simulink model "Model"  (R2016a)
settings: Solver=VariableStepAuto  StartTime=0.0  StopTime=0  RelTol=1e-3
values from neighbouring files (symbols this model uses):
  disdef = variable(a, 7)    [CollectionAG806_808.m]
  Dpha = 0    [CollectionAG806_808.m]    (also in CourantCCabc.m)
  Dphb = -120    [CollectionAG806_808.m]    (also in CourantCCabc.m)
  Dphc = +120    (= 120)    [CollectionAG806_808.m]    (also in CourantCCabc.m)
  frequence = 60    [CollectionAG806_808.m]    (also in CourantCCabc.m)
  Qc844 = [100e3 100e3 100e3]    [CollectionAG806_808.m]    (also in CourantCCabc.m)
  Qc848 = [150e3 150e3 150e3]    [CollectionAG806_808.m]    (also in CourantCCabc.m)
  RF1 = variable(a, 6)    [CollectionAG806_808.m]
  Ustation = variable(a, 2)    [CollectionAG806_808.m]
  Vstation = variable(a, 1)    [CollectionAG806_808.m]
undefined symbols (not defined in the file or in its folder): activeA, activeB, activeC, C_300, C_301, C_302, C_303, C_304, L_300, L_301, L_302, L_303, L_304, Ltot_806_808, R_300, R_301, R_302, R_303, R_304, reactiveA, reactiveB, reactiveC
libraries: powerlib x311
(part 1 of 2)
settings Model: Creator=HP  LastModifiedBy=HP

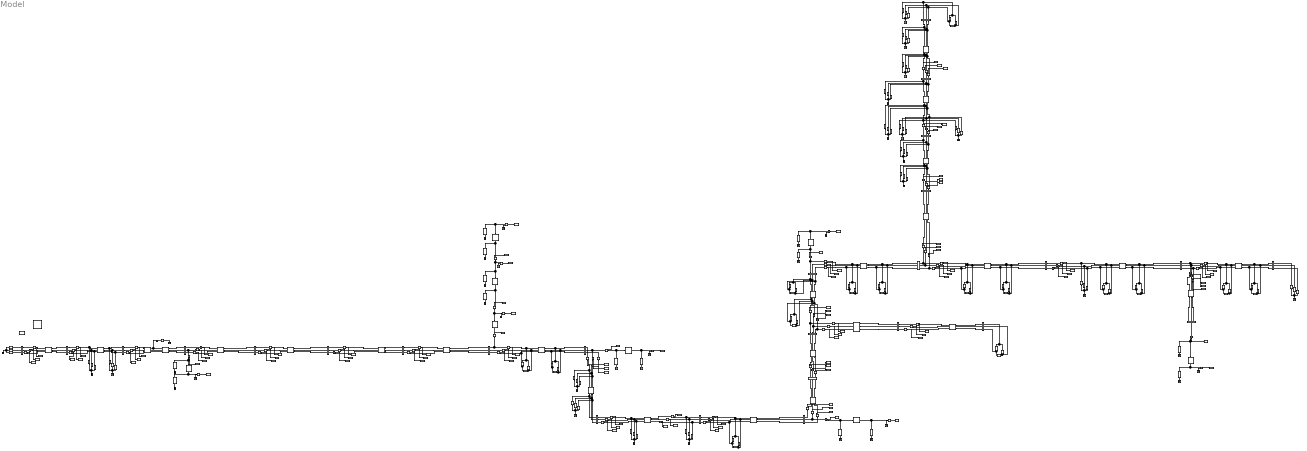
== system Model ==
  "800 " : powerlib/Measurements/Three-Phase V-I Measurement  VoltageMeasurement=phase-to-ground  SetLabelV=on  LabelV=V800  Vpu=off  VpuLL=off  CurrentMeasurement=no  SetLabelI=on  LabelI=I800_802  Ipu=off  Pbase=100e6  Vbase=500e3  OutputType=Complex  PhasorSimulation=on  PSBequivalent=0
  "802 " : powerlib/Measurements/Three-Phase V-I Measurement  VoltageMeasurement=phase-to-ground  SetLabelV=on  LabelV=V802  Vpu=off  VpuLL=off  CurrentMeasurement=no  SetLabelI=on  LabelI=I802_806  Ipu=off  Pbase=100e6  Vbase=500e3  OutputType=Complex  PhasorSimulation=on  PSBequivalent=0
  806 : powerlib/Measurements/Three-Phase V-I Measurement  VoltageMeasurement=phase-to-ground  SetLabelV=on  LabelV=V806  Vpu=off  VpuLL=off  CurrentMeasurement=no  SetLabelI=on  LabelI=I806_808  Ipu=off  Pbase=100e6  Vbase=500e3  OutputType=Complex  PhasorSimulation=on  PSBequivalent=0
  808 : powerlib/Measurements/Three-Phase V-I Measurement  VoltageMeasurement=phase-to-ground  SetLabelV=on  LabelV=V808  Vpu=off  VpuLL=off  CurrentMeasurement=no  SetLabelI=on  LabelI=I808_810_812  Ipu=off  Pbase=100e6  Vbase=500e3  OutputType=Complex  PhasorSimulation=on  PSBequivalent=0
  812 : powerlib/Measurements/Three-Phase V-I Measurement  VoltageMeasurement=phase-to-ground  SetLabelV=on  LabelV=V812  Vpu=off  VpuLL=off  CurrentMeasurement=no  SetLabelI=on  LabelI=I812_814  Ipu=off  Pbase=100e6  Vbase=500e3  OutputType=Complex  PhasorSimulation=on  PSBequivalent=0
  814 : powerlib/Measurements/Three-Phase V-I Measurement  VoltageMeasurement=phase-to-ground  SetLabelV=on  LabelV=V814  Vpu=off  VpuLL=off  CurrentMeasurement=no  SetLabelI=on  LabelI=I814_850  Ipu=off  Pbase=100e6  Vbase=500e3  OutputType=Complex  PhasorSimulation=on  PSBequivalent=0
  816 : powerlib/Measurements/Three-Phase V-I Measurement  VoltageMeasurement=phase-to-ground  SetLabelV=on  LabelV=V816  Vpu=off  VpuLL=off  CurrentMeasurement=no  SetLabelI=on  LabelI=I816_818_824  Ipu=off  Pbase=100e6  Vbase=500e3  OutputType=Complex  PhasorSimulation=on  PSBequivalent=0
  824 : powerlib/Measurements/Three-Phase V-I Measurement  VoltageMeasurement=phase-to-ground  SetLabelV=on  LabelV=V824  Vpu=off  VpuLL=off  CurrentMeasurement=no  SetLabelI=on  LabelI=I824_826_828  Ipu=off  Pbase=100e6  Vbase=500e3  OutputType=Complex  PhasorSimulation=on  PSBequivalent=0
  828 : powerlib/Measurements/Three-Phase V-I Measurement  VoltageMeasurement=phase-to-ground  SetLabelV=on  LabelV=V828  Vpu=off  VpuLL=off  CurrentMeasurement=no  SetLabelI=on  LabelI=I828_830  Ipu=off  Pbase=100e6  Vbase=500e3  OutputType=Complex  PhasorSimulation=on  PSBequivalent=0
  830 : powerlib/Measurements/Three-Phase V-I Measurement  VoltageMeasurement=phase-to-ground  SetLabelV=on  LabelV=V830  Vpu=off  VpuLL=off  CurrentMeasurement=no  SetLabelI=on  LabelI=I830_854  Ipu=off  Pbase=100e6  Vbase=500e3  OutputType=Complex  PhasorSimulation=on  PSBequivalent=0
  832 : powerlib/Measurements/Three-Phase V-I Measurement  VoltageMeasurement=phase-to-ground  SetLabelV=on  LabelV=V832  Vpu=off  VpuLL=off  CurrentMeasurement=no  SetLabelI=on  LabelI=I832_858_888  Ipu=off  Pbase=100e6  Vbase=500e3  OutputType=Complex  PhasorSimulation=on  PSBequivalent=0
  834 : powerlib/Measurements/Three-Phase V-I Measurement  VoltageMeasurement=phase-to-ground  SetLabelV=on  LabelV=V834  Vpu=off  VpuLL=off  CurrentMeasurement=no  SetLabelI=off  LabelI=I834_842_860  Ipu=off  Pbase=100e6  Vbase=500e3  OutputType=Complex  PhasorSimulation=on  PSBequivalent=0
  836 : powerlib/Measurements/Three-Phase V-I Measurement  VoltageMeasurement=phase-to-ground  SetLabelV=on  LabelV=V836  Vpu=off  VpuLL=off  CurrentMeasurement=no  SetLabelI=off  LabelI=Iabc  Ipu=off  Pbase=100e6  Vbase=500e3  OutputType=Complex  PhasorSimulation=on  PSBequivalent=0
  840 : powerlib/Measurements/Three-Phase V-I Measurement  VoltageMeasurement=phase-to-ground  SetLabelV=on  LabelV=V840  Vpu=off  VpuLL=off  CurrentMeasurement=no  SetLabelI=on  LabelI=Iabc  Ipu=off  Pbase=100e6  Vbase=500e3  OutputType=Complex  PhasorSimulation=on  PSBequivalent=0
  842 : powerlib/Measurements/Three-Phase V-I Measurement  VoltageMeasurement=phase-to-ground  SetLabelV=on  LabelV=V842  Vpu=off  VpuLL=off  CurrentMeasurement=no  SetLabelI=on  LabelI=I842_844  Ipu=off  Pbase=100e6  Vbase=500e3  OutputType=Complex  PhasorSimulation=on  PSBequivalent=0
  844 : powerlib/Measurements/Three-Phase V-I Measurement  VoltageMeasurement=phase-to-ground  SetLabelV=on  LabelV=V844  Vpu=off  VpuLL=off  CurrentMeasurement=no  SetLabelI=on  LabelI=I844_846  Ipu=off  Pbase=100e6  Vbase=500e3  OutputType=Complex  PhasorSimulation=on  PSBequivalent=0
  846 : powerlib/Measurements/Three-Phase V-I Measurement  VoltageMeasurement=phase-to-ground  SetLabelV=on  LabelV=V846  Vpu=off  VpuLL=off  CurrentMeasurement=no  SetLabelI=on  LabelI=I846_848  Ipu=off  Pbase=100e6  Vbase=500e3  OutputType=Complex  PhasorSimulation=on  PSBequivalent=0
  848 : powerlib/Measurements/Three-Phase V-I Measurement  VoltageMeasurement=phase-to-ground  SetLabelV=on  LabelV=V848  Vpu=off  VpuLL=off  CurrentMeasurement=no  SetLabelI=on  LabelI=I846_848  Ipu=off  Pbase=100e6  Vbase=500e3  OutputType=Complex  PhasorSimulation=on  PSBequivalent=0
  850 : powerlib/Measurements/Three-Phase V-I Measurement  VoltageMeasurement=phase-to-ground  SetLabelV=on  LabelV=V850  Vpu=off  VpuLL=off  CurrentMeasurement=no  SetLabelI=on  LabelI=I850_816  Ipu=off  Pbase=100e6  Vbase=500e3  OutputType=Complex  PhasorSimulation=on  PSBequivalent=0
  852 : powerlib/Measurements/Three-Phase V-I Measurement  VoltageMeasurement=phase-to-ground  SetLabelV=on  LabelV=V852  Vpu=off  VpuLL=off  CurrentMeasurement=no  SetLabelI=on  LabelI=I852_832  Ipu=off  Pbase=100e6  Vbase=500e3  OutputType=Complex  PhasorSimulation=on  PSBequivalent=0
  854 : powerlib/Measurements/Three-Phase V-I Measurement  VoltageMeasurement=phase-to-ground  SetLabelV=on  LabelV=V854  Vpu=off  VpuLL=off  CurrentMeasurement=no  SetLabelI=on  LabelI=I854_852_856  Ipu=off  Pbase=100e6  Vbase=500e3  OutputType=Complex  PhasorSimulation=on  PSBequivalent=0
  858 : powerlib/Measurements/Three-Phase V-I Measurement  VoltageMeasurement=phase-to-ground  SetLabelV=on  LabelV=V858  Vpu=off  VpuLL=off  CurrentMeasurement=no  SetLabelI=on  LabelI=I858_834_864  Ipu=off  Pbase=100e6  Vbase=500e3  OutputType=Complex  PhasorSimulation=on  PSBequivalent=0
  860 : powerlib/Measurements/Three-Phase V-I Measurement  VoltageMeasurement=phase-to-ground  SetLabelV=on  LabelV=V860  Vpu=off  VpuLL=off  CurrentMeasurement=no  SetLabelI=on  LabelI=I860_836  Ipu=off  Pbase=100e6  Vbase=500e3  OutputType=Complex  PhasorSimulation=on  PSBequivalent=0
  862 : powerlib/Measurements/Three-Phase V-I Measurement  VoltageMeasurement=phase-to-ground  SetLabelV=on  LabelV=V862  Vpu=off  VpuLL=off  CurrentMeasurement=no  SetLabelI=on  LabelI=Iabc  Ipu=off  Pbase=100e6  Vbase=500e3  OutputType=Complex  PhasorSimulation=on  PSBequivalent=0
  888 : powerlib/Measurements/Three-Phase V-I Measurement  VoltageMeasurement=phase-to-ground  SetLabelV=on  LabelV=V888  Vpu=off  VpuLL=off  CurrentMeasurement=no  SetLabelI=on  LabelI=I888_890  Ipu=off  Pbase=100e6  Vbase=500e3  OutputType=Complex  PhasorSimulation=on  PSBequivalent=0
  890 : powerlib/Measurements/Three-Phase V-I Measurement  VoltageMeasurement=phase-to-ground  SetLabelV=on  LabelV=V890  Vpu=off  VpuLL=off  CurrentMeasurement=no  SetLabelI=on  LabelI=I888_890  Ipu=off  Pbase=100e6  Vbase=500e3  OutputType=Complex  PhasorSimulation=on  PSBequivalent=0
  Breaker : powerlib/Elements/Breaker  InitialState=0  SwitchingTimes=0  External=off  BreakerResistance=0.01  SnubberResistance=1e6  SnubberCapacitance=inf  Measurements=None  MoreParameters=on  NoBreakLoop=off
  Ground{,1..40} (41 alike) : powerlib/Elements/Ground  LConnTagsString=a
  Ia800_802 : powerlib/Measurements/Current Measurement  PhasorSimulation=on  OutputType=Complex  PSBequivalent=0
  Ia802_806 : powerlib/Measurements/Current Measurement  PhasorSimulation=on  OutputType=Complex  PSBequivalent=0
  Ia806_808 : powerlib/Measurements/Current Measurement  PhasorSimulation=on  OutputType=Complex  PSBequivalent=0
  Ia808_812 : powerlib/Measurements/Current Measurement  PhasorSimulation=on  OutputType=Complex  PSBequivalent=0
  Ia812_814 : powerlib/Measurements/Current Measurement  PhasorSimulation=on  OutputType=Complex  PSBequivalent=0
  Ia814_850 : powerlib/Measurements/Current Measurement  PhasorSimulation=on  OutputType=Complex  PSBequivalent=0
  Ia816_818 : powerlib/Measurements/Current Measurement  PhasorSimulation=on  OutputType=Complex  PSBequivalent=0
  Ia816_824 : powerlib/Measurements/Current Measurement  PhasorSimulation=on  OutputType=Complex  PSBequivalent=0
  Ia818_820 : powerlib/Measurements/Current Measurement  PhasorSimulation=on  OutputType=Complex  PSBequivalent=0
  Ia820_822 : powerlib/Measurements/Current Measurement  PhasorSimulation=on  OutputType=Complex  PSBequivalent=0
  Ia824_828 : powerlib/Measurements/Current Measurement  PhasorSimulation=on  OutputType=Complex  PSBequivalent=0
  Ia828_830 : powerlib/Measurements/Current Measurement  PhasorSimulation=on  OutputType=Complex  PSBequivalent=0
  Ia830_1 : powerlib/Measurements/Current Measurement  PhasorSimulation=on  OutputType=Complex  PSBequivalent=0
  Ia830_854 : powerlib/Measurements/Current Measurement  PhasorSimulation=on  OutputType=Complex  PSBequivalent=0
  Ia832_858 : powerlib/Measurements/Current Measurement  PhasorSimulation=on  OutputType=Complex  PSBequivalent=0
  Ia832_888 : powerlib/Measurements/Current Measurement  PhasorSimulation=on  OutputType=Complex  PSBequivalent=0
  Ia834_842 : powerlib/Measurements/Current Measurement  PhasorSimulation=on  OutputType=Complex  PSBequivalent=0
  Ia834_860 : powerlib/Measurements/Current Measurement  PhasorSimulation=on  OutputType=Complex  PSBequivalent=0
  Ia836_840 : powerlib/Measurements/Current Measurement  PhasorSimulation=on  OutputType=Complex  PSBequivalent=0
  Ia836_862 : powerlib/Measurements/Current Measurement  PhasorSimulation=on  OutputType=Complex  PSBequivalent=0
  Ia842_844 : powerlib/Measurements/Current Measurement  PhasorSimulation=on  OutputType=Complex  PSBequivalent=0
  Ia844_846 : powerlib/Measurements/Current Measurement  PhasorSimulation=on  OutputType=Complex  PSBequivalent=0
  Ia846_848 : powerlib/Measurements/Current Measurement  PhasorSimulation=on  OutputType=Complex  PSBequivalent=0
  Ia850_816 : powerlib/Measurements/Current Measurement  PhasorSimulation=on  OutputType=Complex  PSBequivalent=0
  Ia852_832 : powerlib/Measurements/Current Measurement  PhasorSimulation=on  OutputType=Complex  PSBequivalent=0
  Ia854_852 : powerlib/Measurements/Current Measurement  PhasorSimulation=on  OutputType=Complex  PSBequivalent=0
  Ia858_834 : powerlib/Measurements/Current Measurement  PhasorSimulation=on  OutputType=Complex  PSBequivalent=0
  Ia858_864 : powerlib/Measurements/Current Measurement  PhasorSimulation=on  OutputType=Complex  PSBequivalent=0
  Ia860_836 : powerlib/Measurements/Current Measurement  PhasorSimulation=on  OutputType=Complex  PSBequivalent=0
  Ia888_890 : powerlib/Measurements/Current Measurement  PhasorSimulation=on  OutputType=Complex  PSBequivalent=0
  Ib800_802 : powerlib/Measurements/Current Measurement  PhasorSimulation=on  OutputType=Complex  PSBequivalent=0
  Ib802_806 : powerlib/Measurements/Current Measurement  PhasorSimulation=on  OutputType=Complex  PSBequivalent=0
  Ib806_808 : powerlib/Measurements/Current Measurement  PhasorSimulation=on  OutputType=Complex  PSBequivalent=0
  Ib808_810 : powerlib/Measurements/Current Measurement  PhasorSimulation=on  OutputType=Complex  PSBequivalent=0
  Ib808_812 : powerlib/Measurements/Current Measurement  PhasorSimulation=on  OutputType=Complex  PSBequivalent=0
  Ib812_814 : powerlib/Measurements/Current Measurement  PhasorSimulation=on  OutputType=Complex  PSBequivalent=0
  Ib814_850 : powerlib/Measurements/Current Measurement  PhasorSimulation=on  OutputType=Complex  PSBequivalent=0
  Ib816_824 : powerlib/Measurements/Current Measurement  PhasorSimulation=on  OutputType=Complex  PSBequivalent=0
  Ib824_826 : powerlib/Measurements/Current Measurement  PhasorSimulation=on  OutputType=Complex  PSBequivalent=0
  Ib824_828 : powerlib/Measurements/Current Measurement  PhasorSimulation=on  OutputType=Complex  PSBequivalent=0
  Ib828_830 : powerlib/Measurements/Current Measurement  PhasorSimulation=on  OutputType=Complex  PSBequivalent=0
  Ib830_1 : powerlib/Measurements/Current Measurement  PhasorSimulation=on  OutputType=Complex  PSBequivalent=0
  Ib830_854 : powerlib/Measurements/Current Measurement  PhasorSimulation=on  OutputType=Complex  PSBequivalent=0
  Ib832_858 : powerlib/Measurements/Current Measurement  PhasorSimulation=on  OutputType=Complex  PSBequivalent=0
  Ib832_888 : powerlib/Measurements/Current Measurement  PhasorSimulation=on  OutputType=Complex  PSBequivalent=0
  Ib834_842 : powerlib/Measurements/Current Measurement  PhasorSimulation=on  OutputType=Complex  PSBequivalent=0
  Ib834_860 : powerlib/Measurements/Current Measurement  PhasorSimulation=on  OutputType=Complex  PSBequivalent=0
  Ib836_840 : powerlib/Measurements/Current Measurement  PhasorSimulation=on  OutputType=Complex  PSBequivalent=0
  Ib836_862 : powerlib/Measurements/Current Measurement  PhasorSimulation=on  OutputType=Complex  PSBequivalent=0
  Ib842_844 : powerlib/Measurements/Current Measurement  PhasorSimulation=on  OutputType=Complex  PSBequivalent=0
  Ib846_846 : powerlib/Measurements/Current Measurement  PhasorSimulation=on  OutputType=Complex  PSBequivalent=0
  Ib846_848 : powerlib/Measurements/Current Measurement  PhasorSimulation=on  OutputType=Complex  PSBequivalent=0
  Ib850_816 : powerlib/Measurements/Current Measurement  PhasorSimulation=on  OutputType=Complex  PSBequivalent=0
  Ib852_832 : powerlib/Measurements/Current Measurement  PhasorSimulation=on  OutputType=Complex  PSBequivalent=0
  Ib854_852 : powerlib/Measurements/Current Measurement  PhasorSimulation=on  OutputType=Complex  PSBequivalent=0
  Ib854_856 : powerlib/Measurements/Current Measurement  PhasorSimulation=on  OutputType=Complex  PSBequivalent=0
  Ib858_834 : powerlib/Measurements/Current Measurement  PhasorSimulation=on  OutputType=Complex  PSBequivalent=0
  Ib860_836 : powerlib/Measurements/Current Measurement  PhasorSimulation=on  OutputType=Complex  PSBequivalent=0
  Ib862_838 : powerlib/Measurements/Current Measurement  PhasorSimulation=on  OutputType=Complex  PSBequivalent=0
  Ib888_890 : powerlib/Measurements/Current Measurement  PhasorSimulation=on  OutputType=Complex  PSBequivalent=0
  Ic800_802 : powerlib/Measurements/Current Measurement  PhasorSimulation=on  OutputType=Complex  PSBequivalent=0
  Ic802_806 : powerlib/Measurements/Current Measurement  PhasorSimulation=on  OutputType=Complex  PSBequivalent=0
  Ic806_808 : powerlib/Measurements/Current Measurement  PhasorSimulation=on  OutputType=Complex  PSBequivalent=0
  Ic808_812 : powerlib/Measurements/Current Measurement  PhasorSimulation=on  OutputType=Complex  PSBequivalent=0
  Ic812_814 : powerlib/Measurements/Current Measurement  PhasorSimulation=on  OutputType=Complex  PSBequivalent=0
  Ic814_850 : powerlib/Measurements/Current Measurement  PhasorSimulation=on  OutputType=Complex  PSBequivalent=0
  Ic816_824 : powerlib/Measurements/Current Measurement  PhasorSimulation=on  OutputType=Complex  PSBequivalent=0
  Ic824_828 : powerlib/Measurements/Current Measurement  PhasorSimulation=on  OutputType=Complex  PSBequivalent=0
  Ic828_830 : powerlib/Measurements/Current Measurement  PhasorSimulation=on  OutputType=Complex  PSBequivalent=0
  Ic830_1 : powerlib/Measurements/Current Measurement  PhasorSimulation=on  OutputType=Complex  PSBequivalent=0
  Ic830_854 : powerlib/Measurements/Current Measurement  PhasorSimulation=on  OutputType=Complex  PSBequivalent=0
  Ic832_858 : powerlib/Measurements/Current Measurement  PhasorSimulation=on  OutputType=Complex  PSBequivalent=0
  Ic832_888 : powerlib/Measurements/Current Measurement  PhasorSimulation=on  OutputType=Complex  PSBequivalent=0
  Ic834_842 : powerlib/Measurements/Current Measurement  PhasorSimulation=on  OutputType=Complex  PSBequivalent=0
  Ic834_860 : powerlib/Measurements/Current Measurement  PhasorSimulation=on  OutputType=Complex  PSBequivalent=0
  Ic836_840 : powerlib/Measurements/Current Measurement  PhasorSimulation=on  OutputType=Complex  PSBequivalent=0
  Ic836_862 : powerlib/Measurements/Current Measurement  PhasorSimulation=on  OutputType=Complex  PSBequivalent=0
  Ic842_844 : powerlib/Measurements/Current Measurement  PhasorSimulation=on  OutputType=Complex  PSBequivalent=0
  Ic844_846 : powerlib/Measurements/Current Measurement  PhasorSimulation=on  OutputType=Complex  PSBequivalent=0
  Ic846_848 : powerlib/Measurements/Current Measurement  PhasorSimulation=on  OutputType=Complex  PSBequivalent=0
  Ic850_816 : powerlib/Measurements/Current Measurement  PhasorSimulation=on  OutputType=Complex  PSBequivalent=0
  Ic852_832 : powerlib/Measurements/Current Measurement  PhasorSimulation=on  OutputType=Complex  PSBequivalent=0
  "Ic854_852 " : powerlib/Measurements/Current Measurement  PhasorSimulation=on  OutputType=Complex  PSBequivalent=0
  Ic858_834 : powerlib/Measurements/Current Measurement  PhasorSimulation=on  OutputType=Complex  PSBequivalent=0
  Ic860_836 : powerlib/Measurements/Current Measurement  PhasorSimulation=on  OutputType=Complex  PSBequivalent=0
  Ic888_890 : powerlib/Measurements/Current Measurement  PhasorSimulation=on  OutputType=Complex  PSBequivalent=0
  RF1 : powerlib/Elements/Series RLC Branch  LConnTagsString=__new0  RConnTagsString=__new0  BranchType=R  Resistance=RF1  Inductance=1e-3  SetiL0=off  InitialCurrent=0  Capacitance=1e-6  Setx0=off  InitialVoltage=0  Measurements=None
  To Workspace : ToWorkspace  VariableName=Ia800_802  SampleTime=-1
      settings: Save2DSignal=2-D array (concatenate along first dimension)
  To Workspace1 : ToWorkspace  VariableName=Ib800_802  SampleTime=-1
      settings: Save2DSignal=2-D array (concatenate along first dimension)
  To Workspace10 : ToWorkspace  VariableName=Ib808_812  SampleTime=-1
      settings: Save2DSignal=2-D array (concatenate along first dimension)
  To Workspace11 : ToWorkspace  VariableName=Ic808_812  SampleTime=-1
      settings: Save2DSignal=2-D array (concatenate along first dimension)
  To Workspace12 : ToWorkspace  VariableName=Ib808_810  SampleTime=-1
      settings: Save2DSignal=2-D array (concatenate along first dimension)
  To Workspace13 : ToWorkspace  VariableName=Ib812_814  SampleTime=-1
      settings: Save2DSignal=2-D array (concatenate along first dimension)
  To Workspace14 : ToWorkspace  VariableName=Ic812_814  SampleTime=-1
      settings: Save2DSignal=2-D array (concatenate along first dimension)
  To Workspace15 : ToWorkspace  VariableName=Ia812_814  SampleTime=-1
      settings: Save2DSignal=2-D array (concatenate along first dimension)
  To Workspace16 : ToWorkspace  VariableName=Ib814_850  SampleTime=-1
      settings: Save2DSignal=2-D array (concatenate along first dimension)
  To Workspace17 : ToWorkspace  VariableName=Ic814_850  SampleTime=-1
      settings: Save2DSignal=2-D array (concatenate along first dimension)
  To Workspace18 : ToWorkspace  VariableName=Ia814_850  SampleTime=-1
      settings: Save2DSignal=2-D array (concatenate along first dimension)
  To Workspace19 : ToWorkspace  VariableName=Ib850_816  SampleTime=-1
      settings: Save2DSignal=2-D array (concatenate along first dimension)
  To Workspace2 : ToWorkspace  VariableName=Ic800_802  SampleTime=-1
      settings: Save2DSignal=2-D array (concatenate along first dimension)
  To Workspace20 : ToWorkspace  VariableName=Ic850_816  SampleTime=-1
      settings: Save2DSignal=2-D array (concatenate along first dimension)
  To Workspace21 : ToWorkspace  VariableName=Ia850_816  SampleTime=-1
      settings: Save2DSignal=2-D array (concatenate along first dimension)
  To Workspace22 : ToWorkspace  VariableName=Ib816_824  SampleTime=-1
      settings: Save2DSignal=2-D array (concatenate along first dimension)
  To Workspace23 : ToWorkspace  VariableName=Ic816_824  SampleTime=-1
      settings: Save2DSignal=2-D array (concatenate along first dimension)
  To Workspace24 : ToWorkspace  VariableName=Ia816_824  SampleTime=-1
      settings: Save2DSignal=2-D array (concatenate along first dimension)
  To Workspace25 : ToWorkspace  VariableName=Ia816_818  SampleTime=-1
      settings: Save2DSignal=2-D array (concatenate along first dimension)
  To Workspace26 : ToWorkspace  VariableName=V818  SampleTime=-1
      settings: Save2DSignal=2-D array (concatenate along first dimension)
  To Workspace27 : ToWorkspace  VariableName=Ia818_820  SampleTime=-1
      settings: Save2DSignal=2-D array (concatenate along first dimension)
  To Workspace28 : ToWorkspace  VariableName=V820  SampleTime=-1
      settings: Save2DSignal=2-D array (concatenate along first dimension)
  To Workspace29 : ToWorkspace  VariableName=Ia820_822  SampleTime=-1
      settings: Save2DSignal=2-D array (concatenate along first dimension)
  To Workspace3 : ToWorkspace  VariableName=Ia802_806  SampleTime=-1
      settings: Save2DSignal=2-D array (concatenate along first dimension)
  To Workspace30 : ToWorkspace  VariableName=Ib824_826  SampleTime=-1
      settings: Save2DSignal=2-D array (concatenate along first dimension)
  To Workspace31 : ToWorkspace  VariableName=Ia824_828  SampleTime=-1
      settings: Save2DSignal=2-D array (concatenate along first dimension)
  To Workspace32 : ToWorkspace  VariableName=Ib824_828  SampleTime=-1
      settings: Save2DSignal=2-D array (concatenate along first dimension)
  To Workspace33 : ToWorkspace  VariableName=Ic824_828  SampleTime=-1
      settings: Save2DSignal=2-D array (concatenate along first dimension)
  To Workspace34 : ToWorkspace  VariableName=Ib828_830  SampleTime=-1
      settings: Save2DSignal=2-D array (concatenate along first dimension)
  To Workspace35 : ToWorkspace  VariableName=Ic828_830  SampleTime=-1
      settings: Save2DSignal=2-D array (concatenate along first dimension)
  To Workspace36 : ToWorkspace  VariableName=Ia828_830  SampleTime=-1
      settings: Save2DSignal=2-D array (concatenate along first dimension)
  To Workspace37 : ToWorkspace  VariableName=Ib830_854  SampleTime=-1
      settings: Save2DSignal=2-D array (concatenate along first dimension)
  To Workspace38 : ToWorkspace  VariableName=Ic830_854  SampleTime=-1
      settings: Save2DSignal=2-D array (concatenate along first dimension)
  To Workspace39 : ToWorkspace  VariableName=Ia830_854  SampleTime=-1
      settings: Save2DSignal=2-D array (concatenate along first dimension)
  To Workspace4 : ToWorkspace  VariableName=Ib802_806  SampleTime=-1
      settings: Save2DSignal=2-D array (concatenate along first dimension)
  To Workspace40 : ToWorkspace  VariableName=Ib854_852  SampleTime=-1
      settings: Save2DSignal=2-D array (concatenate along first dimension)
  To Workspace41 : ToWorkspace  VariableName=Ic854_852  SampleTime=-1
      settings: Save2DSignal=2-D array (concatenate along first dimension)
  To Workspace42 : ToWorkspace  VariableName=Ia854_852  SampleTime=-1
      settings: Save2DSignal=2-D array (concatenate along first dimension)
  To Workspace43 : ToWorkspace  VariableName=Ib854_856  SampleTime=-1
      settings: Save2DSignal=2-D array (concatenate along first dimension)
  To Workspace44 : ToWorkspace  VariableName=Ib852_832  SampleTime=-1
      settings: Save2DSignal=2-D array (concatenate along first dimension)
  To Workspace45 : ToWorkspace  VariableName=Ic852_832  SampleTime=-1
      settings: Save2DSignal=2-D array (concatenate along first dimension)
  To Workspace46 : ToWorkspace  VariableName=Ia852_832  SampleTime=-1
      settings: Save2DSignal=2-D array (concatenate along first dimension)
  To Workspace47 : ToWorkspace  VariableName=Ib832_858  SampleTime=-1
      settings: Save2DSignal=2-D array (concatenate along first dimension)
  To Workspace48 : ToWorkspace  VariableName=Ic832_858  SampleTime=-1
      settings: Save2DSignal=2-D array (concatenate along first dimension)
  To Workspace49 : ToWorkspace  VariableName=Ia832_858  SampleTime=-1
      settings: Save2DSignal=2-D array (concatenate along first dimension)
  To Workspace5 : ToWorkspace  VariableName=Ic802_806  SampleTime=-1
      settings: Save2DSignal=2-D array (concatenate along first dimension)
  To Workspace50 : ToWorkspace  VariableName=Ia858_864  SampleTime=-1
      settings: Save2DSignal=2-D array (concatenate along first dimension)
  To Workspace51 : ToWorkspace  VariableName=Ib832_888  SampleTime=-1
      settings: Save2DSignal=2-D array (concatenate along first dimension)
  To Workspace52 : ToWorkspace  VariableName=Ic832_888  SampleTime=-1
      settings: Save2DSignal=2-D array (concatenate along first dimension)
  To Workspace53 : ToWorkspace  VariableName=Ia832_888  SampleTime=-1
      settings: Save2DSignal=2-D array (concatenate along first dimension)
  To Workspace54 : ToWorkspace  VariableName=Ib888_890  SampleTime=-1
      settings: Save2DSignal=2-D array (concatenate along first dimension)
  To Workspace55 : ToWorkspace  VariableName=Ic888_890  SampleTime=-1
      settings: Save2DSignal=2-D array (concatenate along first dimension)
  To Workspace56 : ToWorkspace  VariableName=Ia888_890  SampleTime=-1
      settings: Save2DSignal=2-D array (concatenate along first dimension)
  To Workspace57 : ToWorkspace  VariableName=Ib858_834  SampleTime=-1
      settings: Save2DSignal=2-D array (concatenate along first dimension)
  To Workspace58 : ToWorkspace  VariableName=Ic858_834  SampleTime=-1
      settings: Save2DSignal=2-D array (concatenate along first dimension)
  To Workspace59 : ToWorkspace  VariableName=Ia858_834  SampleTime=-1
      settings: Save2DSignal=2-D array (concatenate along first dimension)
  To Workspace6 : ToWorkspace  VariableName=Ia806_808  SampleTime=-1
      settings: Save2DSignal=2-D array (concatenate along first dimension)
  To Workspace60 : ToWorkspace  VariableName=Ib834_860  SampleTime=-1
      settings: Save2DSignal=2-D array (concatenate along first dimension)
  To Workspace61 : ToWorkspace  VariableName=Ic834_860  SampleTime=-1
      settings: Save2DSignal=2-D array (concatenate along first dimension)
  To Workspace62 : ToWorkspace  VariableName=Ia834_860  SampleTime=-1
      settings: Save2DSignal=2-D array (concatenate along first dimension)
  To Workspace63 : ToWorkspace  VariableName=Ib834_842  SampleTime=-1
      settings: Save2DSignal=2-D array (concatenate along first dimension)
  To Workspace64 : ToWorkspace  VariableName=Ic834_842  SampleTime=-1
      settings: Save2DSignal=2-D array (concatenate along first dimension)
  To Workspace65 : ToWorkspace  VariableName=Ia834_842  SampleTime=-1
      settings: Save2DSignal=2-D array (concatenate along first dimension)
  To Workspace66 : ToWorkspace  VariableName=Ib842_844  SampleTime=-1
      settings: Save2DSignal=2-D array (concatenate along first dimension)
  To Workspace67 : ToWorkspace  VariableName=Ic842_844  SampleTime=-1
      settings: Save2DSignal=2-D array (concatenate along first dimension)
  To Workspace68 : ToWorkspace  VariableName=Ia842_844  SampleTime=-1
      settings: Save2DSignal=2-D array (concatenate along first dimension)
  To Workspace69 : ToWorkspace  VariableName=Ib844_846  SampleTime=-1
      settings: Save2DSignal=2-D array (concatenate along first dimension)
  To Workspace7 : ToWorkspace  VariableName=Ib806_808  SampleTime=-1
      settings: Save2DSignal=2-D array (concatenate along first dimension)
  To Workspace70 : ToWorkspace  VariableName=Ic844_846  SampleTime=-1
      settings: Save2DSignal=2-D array (concatenate along first dimension)
  To Workspace71 : ToWorkspace  VariableName=Ia844_846  SampleTime=-1
      settings: Save2DSignal=2-D array (concatenate along first dimension)
  To Workspace72 : ToWorkspace  VariableName=Ib846_848  SampleTime=-1
      settings: Save2DSignal=2-D array (concatenate along first dimension)
  To Workspace73 : ToWorkspace  VariableName=Ic846_848  SampleTime=-1
      settings: Save2DSignal=2-D array (concatenate along first dimension)
  To Workspace74 : ToWorkspace  VariableName=Ia846_848  SampleTime=-1
      settings: Save2DSignal=2-D array (concatenate along first dimension)
  To Workspace75 : ToWorkspace  VariableName=Ib860_836  SampleTime=-1
      settings: Save2DSignal=2-D array (concatenate along first dimension)
  To Workspace76 : ToWorkspace  VariableName=Ic860_836  SampleTime=-1
      settings: Save2DSignal=2-D array (concatenate along first dimension)
  To Workspace77 : ToWorkspace  VariableName=Ia860_836  SampleTime=-1
      settings: Save2DSignal=2-D array (concatenate along first dimension)
  To Workspace78 : ToWorkspace  VariableName=Ib836_840  SampleTime=-1
      settings: Save2DSignal=2-D array (concatenate along first dimension)
  To Workspace79 : ToWorkspace  VariableName=Ic836_840  SampleTime=-1
      settings: Save2DSignal=2-D array (concatenate along first dimension)
  To Workspace8 : ToWorkspace  VariableName=Ic806_808  SampleTime=-1
      settings: Save2DSignal=2-D array (concatenate along first dimension)
  To Workspace80 : ToWorkspace  VariableName=Ia836_840  SampleTime=-1
      settings: Save2DSignal=2-D array (concatenate along first dimension)
  To Workspace81 : ToWorkspace  VariableName=Ib836_862  SampleTime=-1
      settings: Save2DSignal=2-D array (concatenate along first dimension)
  To Workspace82 : ToWorkspace  VariableName=Ic836_862  SampleTime=-1
      settings: Save2DSignal=2-D array (concatenate along first dimension)
  To Workspace83 : ToWorkspace  VariableName=Ia836_862  SampleTime=-1
      settings: Save2DSignal=2-D array (concatenate along first dimension)
  To Workspace84 : ToWorkspace  VariableName=Ib862_838  SampleTime=-1
      settings: Save2DSignal=2-D array (concatenate along first dimension)
  To Workspace85 : ToWorkspace  VariableName=V810  SampleTime=-1
      settings: Save2DSignal=2-D array (concatenate along first dimension)
  To Workspace86 : ToWorkspace  VariableName=V856  SampleTime=-1
      settings: Save2DSignal=2-D array (concatenate along first dimension)
  To Workspace87 : ToWorkspace  VariableName=V822  SampleTime=-1
      settings: Save2DSignal=2-D array (concatenate along first dimension)
  To Workspace88 : ToWorkspace  VariableName=V864  SampleTime=-1
      settings: Save2DSignal=2-D array (concatenate along first dimension)
  To Workspace89 : ToWorkspace  VariableName=V826  SampleTime=-1
      settings: Save2DSignal=2-D array (concatenate along first dimension)
  To Workspace9 : ToWorkspace  VariableName=Ia808_812  SampleTime=-1
      settings: Save2DSignal=2-D array (concatenate along first dimension)
  To Workspace90 : ToWorkspace  VariableName=V838  SampleTime=-1
      settings: Save2DSignal=2-D array (concatenate along first dimension)
  To Workspace91 : ToWorkspace  VariableName=Ita830  SampleTime=-1
      settings: Save2DSignal=2-D array (concatenate along first dimension)
  To Workspace92 : ToWorkspace  VariableName=Itb830  SampleTime=-1
      settings: Save2DSignal=2-D array (concatenate along first dimension)
  To Workspace93 : ToWorkspace  VariableName=Itc830  SampleTime=-1
      settings: Save2DSignal=2-D array (concatenate along first dimension)
  V{810,818,820,822,826,838,856,864} (8 alike) : powerlib/Measurements/Voltage Measurement  PhasorSimulation=on  OutputType=Complex  PSBequivalent=0
  Va : powerlib/Electrical Sources/AC Voltage Source  Amplitude=Vstation  Phase=Dpha  Frequency=frequence  SampleTime=0  Measurements=None  BusType=swing  Pref=10e3  Qref=0  Qmin=-inf  Qmax=+inf
  Vb : powerlib/Electrical Sources/AC Voltage Source  Amplitude=Vstation  Phase=Dphb  Frequency=frequence  SampleTime=0  Measurements=None  BusType=swing  Pref=10e3  Qref=0  Qmin=-inf  Qmax=+inf
  Vc : powerlib/Electrical Sources/AC Voltage Source  Amplitude=Vstation  Phase=Dphc  Frequency=frequence  SampleTime=0  Measurements=None  BusType=swing  Pref=10e3  Qref=0  Qmin=-inf  Qmax=+inf
  XFM-1 : powerlib/Elements/Three-Phase Transformer (Two Windings)  Winding1Connection=Yg  Winding2Connection=Yg  CoreType=Three single-phase transformers  SetSaturation=off  Hysteresis=on  DataFile='hysteresis'  SetInitialFlux=on  Measurements=None  UNITS=pu  NominalPower=[ 500e3 , 60 ]  Winding1=[24.9e3 0.019 0.0408]  Winding2=[4.16e3 0.019 0.0408]  Rm=500  Lm=500  L0=0.15201  Saturation=[0 0;0.00014638 0.022251;0.060992 0.028185]  InitialFluxes=[0.014834 -0.014834 0.01298]  MoreParameters=off  BreakLoop=off  DataType=off  TransfoNumber=1
  charge distributive 802-806 Y-PQ (1)-A : powerlib/Elements/Series RLC Load  LConnTagsString=a  RConnTagsString=__new0  NominalVoltage=Vstation  NominalFrequency=frequence  ActivePower=activeA(2,3)/2  InductivePower=reactiveA(2,3)/2  CapacitivePower=0  Setx0=off  InitialVoltage=0  SetiL0=off  InitialCurrent=0  Measurements=None  LoadType=constant Z
  charge distributive 802-806 Y-PQ (1)-B : powerlib/Elements/Series RLC Load  LConnTagsString=a  RConnTagsString=__new0  NominalVoltage=Vstation  NominalFrequency=frequence  ActivePower=activeB(2,3)/2  InductivePower=reactiveB(2,3)/2  CapacitivePower=0  Setx0=off  InitialVoltage=0  SetiL0=off  InitialCurrent=0  Measurements=None  LoadType=constant Z
  charge distributive 802-806 Y-PQ (1)-C : powerlib/Elements/Series RLC Load  LConnTagsString=a  RConnTagsString=__new0  NominalVoltage=Vstation  NominalFrequency=frequence  ActivePower=activeC(2,3)/2  InductivePower=reactiveC(2,3)/2  CapacitivePower=0  Setx0=off  InitialVoltage=0  SetiL0=off  InitialCurrent=0  Measurements=None  LoadType=constant Z
  charge distributive 802-806 Y-PQ (2)-A : powerlib/Elements/Series RLC Load  LConnTagsString=a  RConnTagsString=__new0  NominalVoltage=Vstation  NominalFrequency=frequence  ActivePower=activeA(2,3)/2  InductivePower=reactiveA(2,3)/2  CapacitivePower=0  Setx0=off  InitialVoltage=0  SetiL0=off  InitialCurrent=0  Measurements=None  LoadType=constant Z
  charge distributive 802-806 Y-PQ (2)-B : powerlib/Elements/Series RLC Load  LConnTagsString=a  RConnTagsString=__new0  NominalVoltage=Vstation  NominalFrequency=frequence  ActivePower=activeB(2,3)/2  InductivePower=reactiveB(2,3)/2  CapacitivePower=0  Setx0=off  InitialVoltage=0  SetiL0=off  InitialCurrent=0  Measurements=None  LoadType=constant Z
  charge distributive 802-806 Y-PQ (2)-C : powerlib/Elements/Series RLC Load  LConnTagsString=a  RConnTagsString=__new0  NominalVoltage=Vstation  NominalFrequency=frequence  ActivePower=activeC(2,3)/2  InductivePower=reactiveC(2,3)/2  CapacitivePower=0  Setx0=off  InitialVoltage=0  SetiL0=off  InitialCurrent=0  Measurements=None  LoadType=constant Z
  charge distributive 808-810 Y-I (1) : powerlib/Elements/Series RLC Load  LConnTagsString=a  RConnTagsString=__new0  NominalVoltage=Vstation  NominalFrequency=frequence  ActivePower=activeB(4,5)./2  InductivePower=reactiveB(4,5)./2  CapacitivePower=0  Setx0=off  InitialVoltage=0  SetiL0=off  InitialCurrent=0  Measurements=None  LoadType=constant I
  charge distributive 808-810 Y-I (2) : powerlib/Elements/Series RLC Load  LConnTagsString=a  RConnTagsString=__new0  NominalVoltage=Vstation  NominalFrequency=frequence  ActivePower=activeB(4,5)./2  InductivePower=reactiveB(4,5)./2  CapacitivePower=0  Setx0=off  InitialVoltage=0  SetiL0=off  InitialCurrent=0  Measurements=None  LoadType=constant I
  charge distributive 816-824 D-I (1)-A : powerlib/Elements/Series RLC Load  LConnTagsString=a  RConnTagsString=__new0  NominalVoltage=Ustation  NominalFrequency=frequence  ActivePower=activeA(9,13)/2  InductivePower=reactiveA(9,13)/2  CapacitivePower=0  Setx0=off  InitialVoltage=0  SetiL0=off  InitialCurrent=0  Measurements=None  LoadType=constant Z
  charge distributive 816-824 D-I (1)-B : powerlib/Elements/Series RLC Load  LConnTagsString=a  RConnTagsString=__new0  NominalVoltage=Ustation  NominalFrequency=frequence  ActivePower=activeB(9,13)/2  InductivePower=reactiveB(9,13)/2  CapacitivePower=0  Setx0=off  InitialVoltage=0  SetiL0=off  InitialCurrent=0  Measurements=None  LoadType=constant Z
  charge distributive 816-824 D-I (1)-C : powerlib/Elements/Series RLC Load  LConnTagsString=a  RConnTagsString=__new0  NominalVoltage=Ustation  NominalFrequency=frequence  ActivePower=activeC(9,13)/2  InductivePower=reactiveC(9,13)/2  CapacitivePower=0  Setx0=off  InitialVoltage=0  SetiL0=off  InitialCurrent=0  Measurements=None  LoadType=constant Z
  charge distributive 816-824 D-I (2)-A : powerlib/Elements/Series RLC Load  LConnTagsString=a  RConnTagsString=__new0  NominalVoltage=Ustation  NominalFrequency=frequence  ActivePower=activeA(9,13)/2  InductivePower=reactiveA(9,13)/2  CapacitivePower=0  Setx0=off  InitialVoltage=0  SetiL0=off  InitialCurrent=0  Measurements=None  LoadType=constant Z
  charge distributive 816-824 D-I (2)-B : powerlib/Elements/Series RLC Load  LConnTagsString=a  RConnTagsString=__new0  NominalVoltage=Ustation  NominalFrequency=frequence  ActivePower=activeB(9,13)/2  InductivePower=reactiveB(9,13)/2  CapacitivePower=0  Setx0=off  InitialVoltage=0  SetiL0=off  InitialCurrent=0  Measurements=None  LoadType=constant Z
  charge distributive 816-824 D-I (2)-C : powerlib/Elements/Series RLC Load  LConnTagsString=a  RConnTagsString=__new0  NominalVoltage=Ustation  NominalFrequency=frequence  ActivePower=activeC(9,13)/2  InductivePower=reactiveC(9,13)/2  CapacitivePower=0  Setx0=off  InitialVoltage=0  SetiL0=off  InitialCurrent=0  Measurements=None  LoadType=constant Z
  charge distributive 818-820 Y-Z (1) : powerlib/Elements/Series RLC Load  LConnTagsString=a  RConnTagsString=__new0  NominalVoltage=Vstation  NominalFrequency=frequence  ActivePower=activeA(10,11)./2  InductivePower=reactiveA(10,11)./2  CapacitivePower=0  Setx0=off  InitialVoltage=0  SetiL0=off  InitialCurrent=0  Measurements=None  LoadType=constant Z
  charge distributive 818-820 Y-Z (2) : powerlib/Elements/Series RLC Load  LConnTagsString=a  RConnTagsString=__new0  NominalVoltage=Vstation  NominalFrequency=frequence  ActivePower=activeA(10,11)./2  InductivePower=reactiveA(10,11)./2  CapacitivePower=0  Setx0=off  InitialVoltage=0  SetiL0=off  InitialCurrent=0  Measurements=None  LoadType=constant Z
  charge distributive 820-822 Y-PQ (1) : powerlib/Elements/Series RLC Load  LConnTagsString=a  RConnTagsString=__new0  NominalVoltage=Vstation  NominalFrequency=frequence  ActivePower=activeA(11,12)./2  InductivePower=reactiveA(11,12)./2  CapacitivePower=0  Setx0=off  InitialVoltage=0  SetiL0=off  InitialCurrent=0  Measurements=None  LoadType=constant PQ
  charge distributive 820-822 Y-PQ (2) : powerlib/Elements/Series RLC Load  LConnTagsString=a  RConnTagsString=__new0  NominalVoltage=Vstation  NominalFrequency=frequence  ActivePower=activeA(11,12)./2  InductivePower=reactiveA(11,12)./2  CapacitivePower=0  Setx0=off  InitialVoltage=0  SetiL0=off  InitialCurrent=0  Measurements=None  LoadType=constant PQ
  charge distributive 824-826 Y-I (1) : powerlib/Elements/Series RLC Load  LConnTagsString=a  RConnTagsString=__new0  NominalVoltage=Vstation  NominalFrequency=frequence  ActivePower=activeB(13,14)./2  InductivePower=reactiveB(13,14)./2  CapacitivePower=0  Setx0=off  InitialVoltage=0  SetiL0=off  InitialCurrent=0  Measurements=None  LoadType=constant I
  charge distributive 824-826 Y-I (2) : powerlib/Elements/Series RLC Load  LConnTagsString=a  RConnTagsString=__new0  NominalVoltage=Vstation  NominalFrequency=frequence  ActivePower=activeB(13,14)./2  InductivePower=reactiveB(13,14)./2  CapacitivePower=0  Setx0=off  InitialVoltage=0  SetiL0=off  InitialCurrent=0  Measurements=None  LoadType=constant I
  charge distributive 824-828 Y-PQ (1)-A : powerlib/Elements/Series RLC Load  LConnTagsString=a  RConnTagsString=__new0  NominalVoltage=Vstation  NominalFrequency=frequence  ActivePower=activeA(13,15)/2  InductivePower=reactiveA(13,15)/2  CapacitivePower=0  Setx0=off  InitialVoltage=0  SetiL0=off  InitialCurrent=0  Measurements=None  LoadType=constant Z
  charge distributive 824-828 Y-PQ (1)-B : powerlib/Elements/Series RLC Load  LConnTagsString=a  RConnTagsString=__new0  NominalVoltage=Vstation  NominalFrequency=frequence  ActivePower=activeB(13,15)/2  InductivePower=reactiveB(13,15)/2  CapacitivePower=0  Setx0=off  InitialVoltage=0  SetiL0=off  InitialCurrent=0  Measurements=None  LoadType=constant Z
  charge distributive 824-828 Y-PQ (1)-C : powerlib/Elements/Series RLC Load  LConnTagsString=a  RConnTagsString=__new0  NominalVoltage=Vstation  NominalFrequency=frequence  ActivePower=activeC(13,15)/2  InductivePower=reactiveC(13,15)/2  CapacitivePower=0  Setx0=off  InitialVoltage=0  SetiL0=off  InitialCurrent=0  Measurements=None  LoadType=constant Z
  charge distributive 824-828 Y-PQ (2)-A : powerlib/Elements/Series RLC Load  LConnTagsString=a  RConnTagsString=__new0  NominalVoltage=Vstation  NominalFrequency=frequence  ActivePower=activeA(13,15)/2  InductivePower=reactiveA(13,15)/2  CapacitivePower=0  Setx0=off  InitialVoltage=0  SetiL0=off  InitialCurrent=0  Measurements=None  LoadType=constant Z
  charge distributive 824-828 Y-PQ (2)-B : powerlib/Elements/Series RLC Load  LConnTagsString=a  RConnTagsString=__new0  NominalVoltage=Vstation  NominalFrequency=frequence  ActivePower=activeB(13,15)/2  InductivePower=reactiveB(13,15)/2  CapacitivePower=0  Setx0=off  InitialVoltage=0  SetiL0=off  InitialCurrent=0  Measurements=None  LoadType=constant Z
  charge distributive 824-828 Y-PQ (2)-C : powerlib/Elements/Series RLC Load  LConnTagsString=a  RConnTagsString=__new0  NominalVoltage=Vstation  NominalFrequency=frequence  ActivePower=activeC(13,15)/2  InductivePower=reactiveC(13,15)/2  CapacitivePower=0  Setx0=off  InitialVoltage=0  SetiL0=off  InitialCurrent=0  Measurements=None  LoadType=constant Z
  charge distributive 828-830 Y-PQ (1)-A : powerlib/Elements/Series RLC Load  LConnTagsString=a  RConnTagsString=__new0  NominalVoltage=Vstation  NominalFrequency=frequence  ActivePower=activeA(15,16)/2  InductivePower=reactiveA(15,16)/2  CapacitivePower=0  Setx0=off  InitialVoltage=0  SetiL0=off  InitialCurrent=0  Measurements=None  LoadType=constant Z
  charge distributive 828-830 Y-PQ (1)-B : powerlib/Elements/Series RLC Load  LConnTagsString=a  RConnTagsString=__new0  NominalVoltage=Vstation  NominalFrequency=frequence  ActivePower=activeB(15,16)/2  InductivePower=reactiveB(15,16)/2  CapacitivePower=0  Setx0=off  InitialVoltage=0  SetiL0=off  InitialCurrent=0  Measurements=None  LoadType=constant Z
  charge distributive 828-830 Y-PQ (1)-C : powerlib/Elements/Series RLC Load  LConnTagsString=a  RConnTagsString=__new0  NominalVoltage=Vstation  NominalFrequency=frequence  ActivePower=activeC(15,16)/2  InductivePower=reactiveC(15,16)/2  CapacitivePower=0  Setx0=off  InitialVoltage=0  SetiL0=off  InitialCurrent=0  Measurements=None  LoadType=constant Z
  charge distributive 828-830 Y-PQ (2)-A : powerlib/Elements/Series RLC Load  LConnTagsString=a  RConnTagsString=__new0  NominalVoltage=Vstation  NominalFrequency=frequence  ActivePower=activeA(15,16)/2  InductivePower=reactiveA(15,16)/2  CapacitivePower=0  Setx0=off  InitialVoltage=0  SetiL0=off  InitialCurrent=0  Measurements=None  LoadType=constant Z
  charge distributive 828-830 Y-PQ (2)-B : powerlib/Elements/Series RLC Load  LConnTagsString=a  RConnTagsString=__new0  NominalVoltage=Vstation  NominalFrequency=frequence  ActivePower=activeB(15,16)/2  InductivePower=reactiveB(15,16)/2  CapacitivePower=0  Setx0=off  InitialVoltage=0  SetiL0=off  InitialCurrent=0  Measurements=None  LoadType=constant Z
  charge distributive 828-830 Y-PQ (2)-C : powerlib/Elements/Series RLC Load  LConnTagsString=a  RConnTagsString=__new0  NominalVoltage=Vstation  NominalFrequency=frequence  ActivePower=activeC(15,16)/2  InductivePower=reactiveC(15,16)/2  CapacitivePower=0  Setx0=off  InitialVoltage=0  SetiL0=off  InitialCurrent=0  Measurements=None  LoadType=constant Z
  charge distributive 832-858 D-Z (1)-A : powerlib/Elements/Series RLC Load  LConnTagsString=a  RConnTagsString=__new0  NominalVoltage=Ustation  NominalFrequency=frequence  ActivePower=activeA(20,23)/2  InductivePower=reactiveA(20,23)/2  CapacitivePower=0  Setx0=off  InitialVoltage=0  SetiL0=off  InitialCurrent=0  Measurements=None  LoadType=constant Z
  charge distributive 832-858 D-Z (1)-B : powerlib/Elements/Series RLC Load  LConnTagsString=a  RConnTagsString=__new0  NominalVoltage=Ustation  NominalFrequency=frequence  ActivePower=activeB(20,23)/2  InductivePower=reactiveB(20,23)/2  CapacitivePower=0  Setx0=off  InitialVoltage=0  SetiL0=off  InitialCurrent=0  Measurements=None  LoadType=constant Z
  charge distributive 832-858 D-Z (1)-C : powerlib/Elements/Series RLC Load  LConnTagsString=a  RConnTagsString=__new0  NominalVoltage=Ustation  NominalFrequency=frequence  ActivePower=activeC(20,23)/2  InductivePower=reactiveC(20,23)/2  CapacitivePower=0  Setx0=off  InitialVoltage=0  SetiL0=off  InitialCurrent=0  Measurements=None  LoadType=constant Z
  charge distributive 832-858 D-Z (2)-A : powerlib/Elements/Series RLC Load  LConnTagsString=a  RConnTagsString=__new0  NominalVoltage=Ustation  NominalFrequency=frequence  ActivePower=activeA(20,23)/2  InductivePower=reactiveA(20,23)/2  CapacitivePower=0  Setx0=off  InitialVoltage=0  SetiL0=off  InitialCurrent=0  Measurements=None  LoadType=constant Z
  charge distributive 832-858 D-Z (2)-B : powerlib/Elements/Series RLC Load  LConnTagsString=a  RConnTagsString=__new0  NominalVoltage=Ustation  NominalFrequency=frequence  ActivePower=activeB(20,23)/2  InductivePower=reactiveB(20,23)/2  CapacitivePower=0  Setx0=off  InitialVoltage=0  SetiL0=off  InitialCurrent=0  Measurements=None  LoadType=constant Z
  charge distributive 832-858 D-Z (2)-C : powerlib/Elements/Series RLC Load  LConnTagsString=a  RConnTagsString=__new0  NominalVoltage=Ustation  NominalFrequency=frequence  ActivePower=activeC(20,23)/2  InductivePower=reactiveC(20,23)/2  CapacitivePower=0  Setx0=off  InitialVoltage=0  SetiL0=off  InitialCurrent=0  Measurements=None  LoadType=constant Z
  charge distributive 834-860 D-Z (1)-A : powerlib/Elements/Series RLC Load  LConnTagsString=a  RConnTagsString=__new0  NominalVoltage=Ustation  NominalFrequency=frequence  ActivePower=activeA(25,30)/2  InductivePower=reactiveA(25,30)/2  CapacitivePower=0  Setx0=off  InitialVoltage=0  SetiL0=off  InitialCurrent=0  Measurements=None  LoadType=constant Z
  charge distributive 834-860 D-Z (1)-B : powerlib/Elements/Series RLC Load  LConnTagsString=a  RConnTagsString=__new0  NominalVoltage=Ustation  NominalFrequency=frequence  ActivePower=activeB(25,30)/2  InductivePower=reactiveB(25,30)/2  CapacitivePower=0  Setx0=off  InitialVoltage=0  SetiL0=off  InitialCurrent=0  Measurements=None  LoadType=constant Z
  charge distributive 834-860 D-Z (1)-C : powerlib/Elements/Series RLC Load  LConnTagsString=a  RConnTagsString=__new0  NominalVoltage=Ustation  NominalFrequency=frequence  ActivePower=activeC(25,30)/2  InductivePower=reactiveC(25,30)/2  CapacitivePower=0  Setx0=off  InitialVoltage=0  SetiL0=off  InitialCurrent=0  Measurements=None  LoadType=constant Z
  charge distributive 834-860 D-Z (2)-A : powerlib/Elements/Series RLC Load  LConnTagsString=a  RConnTagsString=__new0  NominalVoltage=Ustation  NominalFrequency=frequence  ActivePower=activeA(25,30)/2  InductivePower=reactiveA(25,30)/2  CapacitivePower=0  Setx0=off  InitialVoltage=0  SetiL0=off  InitialCurrent=0  Measurements=None  LoadType=constant Z
  charge distributive 834-860 D-Z (2)-B : powerlib/Elements/Series RLC Load  LConnTagsString=a  RConnTagsString=__new0  NominalVoltage=Ustation  NominalFrequency=frequence  ActivePower=activeB(25,30)/2  InductivePower=reactiveB(25,30)/2  CapacitivePower=0  Setx0=off  InitialVoltage=0  SetiL0=off  InitialCurrent=0  Measurements=None  LoadType=constant Z
  charge distributive 834-860 D-Z (2)-C : powerlib/Elements/Series RLC Load  LConnTagsString=a  RConnTagsString=__new0  NominalVoltage=Ustation  NominalFrequency=frequence  ActivePower=activeC(25,30)/2  InductivePower=reactiveC(25,30)/2  CapacitivePower=0  Setx0=off  InitialVoltage=0  SetiL0=off  InitialCurrent=0  Measurements=None  LoadType=constant Z
  charge distributive 836-840 D-I (1)-A : powerlib/Elements/Series RLC Load  LConnTagsString=a  RConnTagsString=__new0  NominalVoltage=Ustation  NominalFrequency=frequence  ActivePower=activeA(31,34)/2  InductivePower=reactiveA(31,34)/2  CapacitivePower=0  Setx0=off  InitialVoltage=0  SetiL0=off  InitialCurrent=0  Measurements=None  LoadType=constant Z
  charge distributive 836-840 D-I (1)-B : powerlib/Elements/Series RLC Load  LConnTagsString=a  RConnTagsString=__new0  NominalVoltage=Ustation  NominalFrequency=frequence  ActivePower=activeB(31,34)/2  InductivePower=reactiveB(31,34)/2  CapacitivePower=0  Setx0=off  InitialVoltage=0  SetiL0=off  InitialCurrent=0  Measurements=None  LoadType=constant Z
  charge distributive 836-840 D-I (1)-C : powerlib/Elements/Series RLC Load  LConnTagsString=a  RConnTagsString=__new0  NominalVoltage=Ustation  NominalFrequency=frequence  ActivePower=activeC(31,34)/2  InductivePower=reactiveC(31,34)/2  CapacitivePower=0  Setx0=off  InitialVoltage=0  SetiL0=off  InitialCurrent=0  Measurements=None  LoadType=constant Z
  charge distributive 836-840 D-I (2)-A : powerlib/Elements/Series RLC Load  LConnTagsString=a  RConnTagsString=__new0  NominalVoltage=Ustation  NominalFrequency=frequence  ActivePower=activeA(31,34)/2  InductivePower=reactiveA(31,34)/2  CapacitivePower=0  Setx0=off  InitialVoltage=0  SetiL0=off  InitialCurrent=0  Measurements=None  LoadType=constant Z
  charge distributive 836-840 D-I (2)-B : powerlib/Elements/Series RLC Load  LConnTagsString=a  RConnTagsString=__new0  NominalVoltage=Ustation  NominalFrequency=frequence  ActivePower=activeB(31,34)/2  InductivePower=reactiveB(31,34)/2  CapacitivePower=0  Setx0=off  InitialVoltage=0  SetiL0=off  InitialCurrent=0  Measurements=None  LoadType=constant Z
  charge distributive 836-840 D-I (2)-C : powerlib/Elements/Series RLC Load  LConnTagsString=a  RConnTagsString=__new0  NominalVoltage=Ustation  NominalFrequency=frequence  ActivePower=activeC(31,34)/2  InductivePower=reactiveC(31,34)/2  CapacitivePower=0  Setx0=off  InitialVoltage=0  SetiL0=off  InitialCurrent=0  Measurements=None  LoadType=constant Z
  charge distributive 842-844 Y-PQ (1)-A : powerlib/Elements/Series RLC Load  LConnTagsString=a  RConnTagsString=__new0  NominalVoltage=Vstation  NominalFrequency=frequence  ActivePower=activeA(26,27)/2  InductivePower=reactiveA(26,27)/2  CapacitivePower=0  Setx0=off  InitialVoltage=0  SetiL0=off  InitialCurrent=0  Measurements=None  LoadType=constant Z
  charge distributive 842-844 Y-PQ (1)-B : powerlib/Elements/Series RLC Load  LConnTagsString=a  RConnTagsString=__new0  NominalVoltage=Vstation  NominalFrequency=frequence  ActivePower=activeB(26,27)/2  InductivePower=reactiveB(26,27)/2  CapacitivePower=0  Setx0=off  InitialVoltage=0  SetiL0=off  InitialCurrent=0  Measurements=None  LoadType=constant Z
  charge distributive 842-844 Y-PQ (1)-C : powerlib/Elements/Series RLC Load  LConnTagsString=a  RConnTagsString=__new0  NominalVoltage=Vstation  NominalFrequency=frequence  ActivePower=activeC(26,27)/2  InductivePower=reactiveC(26,27)/2  CapacitivePower=0  Setx0=off  InitialVoltage=0  SetiL0=off  InitialCurrent=0  Measurements=None  LoadType=constant Z
  charge distributive 842-844 Y-PQ (2)-A : powerlib/Elements/Series RLC Load  LConnTagsString=a  RConnTagsString=__new0  NominalVoltage=Vstation  NominalFrequency=frequence  ActivePower=activeA(26,27)/2  InductivePower=reactiveA(26,27)/2  CapacitivePower=0  Setx0=off  InitialVoltage=0  SetiL0=off  InitialCurrent=0  Measurements=None  LoadType=constant Z
  charge distributive 842-844 Y-PQ (2)-B : powerlib/Elements/Series RLC Load  LConnTagsString=a  RConnTagsString=__new0  NominalVoltage=Vstation  NominalFrequency=frequence  ActivePower=activeB(26,27)/2  InductivePower=reactiveB(26,27)/2  CapacitivePower=0  Setx0=off  InitialVoltage=0  SetiL0=off  InitialCurrent=0  Measurements=None  LoadType=constant Z
  charge distributive 842-844 Y-PQ (2)-C : powerlib/Elements/Series RLC Load  LConnTagsString=a  RConnTagsString=__new0  NominalVoltage=Vstation  NominalFrequency=frequence  ActivePower=activeC(26,27)/2  InductivePower=reactiveC(26,27)/2  CapacitivePower=0  Setx0=off  InitialVoltage=0  SetiL0=off  InitialCurrent=0  Measurements=None  LoadType=constant Z
  charge distributive 844-846 Y-PQ (1)-A : powerlib/Elements/Series RLC Load  LConnTagsString=a  RConnTagsString=__new0  NominalVoltage=Vstation  NominalFrequency=frequence  ActivePower=activeA(27,28)/2  InductivePower=reactiveA(27,28)/2  CapacitivePower=0  Setx0=off  InitialVoltage=0  SetiL0=off  InitialCurrent=0  Measurements=None  LoadType=constant Z
  charge distributive 844-846 Y-PQ (1)-B : powerlib/Elements/Series RLC Load  LConnTagsString=a  RConnTagsString=__new0  NominalVoltage=Vstation  NominalFrequency=frequence  ActivePower=activeB(27,28)/2  InductivePower=reactiveB(27,28)/2  CapacitivePower=0  Setx0=off  InitialVoltage=0  SetiL0=off  InitialCurrent=0  Measurements=None  LoadType=constant Z
  charge distributive 844-846 Y-PQ (1)-C : powerlib/Elements/Series RLC Load  LConnTagsString=a  RConnTagsString=__new0  NominalVoltage=Vstation  NominalFrequency=frequence  ActivePower=activeC(27,28)/2  InductivePower=reactiveC(27,28)/2  CapacitivePower=0  Setx0=off  InitialVoltage=0  SetiL0=off  InitialCurrent=0  Measurements=None  LoadType=constant Z
  charge distributive 844-846 Y-PQ (2)-A : powerlib/Elements/Series RLC Load  LConnTagsString=a  RConnTagsString=__new0  NominalVoltage=Vstation  NominalFrequency=frequence  ActivePower=activeA(27,28)/2  InductivePower=reactiveA(27,28)/2  CapacitivePower=0  Setx0=off  InitialVoltage=0  SetiL0=off  InitialCurrent=0  Measurements=None  LoadType=constant Z
  charge distributive 844-846 Y-PQ (2)-B : powerlib/Elements/Series RLC Load  LConnTagsString=a  RConnTagsString=__new0  NominalVoltage=Vstation  NominalFrequency=frequence  ActivePower=activeB(27,28)/2  InductivePower=reactiveB(27,28)/2  CapacitivePower=0  Setx0=off  InitialVoltage=0  SetiL0=off  InitialCurrent=0  Measurements=None  LoadType=constant Z
  charge distributive 844-846 Y-PQ (2)-C : powerlib/Elements/Series RLC Load  LConnTagsString=a  RConnTagsString=__new0  NominalVoltage=Vstation  NominalFrequency=frequence  ActivePower=activeC(27,28)/2  InductivePower=reactiveC(27,28)/2  CapacitivePower=0  Setx0=off  InitialVoltage=0  SetiL0=off  InitialCurrent=0  Measurements=None  LoadType=constant Z
  charge distributive 846-848 Y-PQ (1)-A : powerlib/Elements/Series RLC Load  LConnTagsString=a  RConnTagsString=__new0  NominalVoltage=Vstation  NominalFrequency=frequence  ActivePower=activeA(28,29)/2  InductivePower=reactiveA(28,29)/2  CapacitivePower=0  Setx0=off  InitialVoltage=0  SetiL0=off  InitialCurrent=0  Measurements=None  LoadType=constant Z
  charge distributive 846-848 Y-PQ (1)-B : powerlib/Elements/Series RLC Load  LConnTagsString=a  RConnTagsString=__new0  NominalVoltage=Vstation  NominalFrequency=frequence  ActivePower=activeB(28,29)/2  InductivePower=reactiveB(28,29)/2  CapacitivePower=0  Setx0=off  InitialVoltage=0  SetiL0=off  InitialCurrent=0  Measurements=None  LoadType=constant Z
  charge distributive 846-848 Y-PQ (1)-C : powerlib/Elements/Series RLC Load  LConnTagsString=a  RConnTagsString=__new0  NominalVoltage=Vstation  NominalFrequency=frequence  ActivePower=activeC(28,29)/2  InductivePower=reactiveC(28,29)/2  CapacitivePower=0  Setx0=off  InitialVoltage=0  SetiL0=off  InitialCurrent=0  Measurements=None  LoadType=constant Z
  charge distributive 846-848 Y-PQ (2)-A : powerlib/Elements/Series RLC Load  LConnTagsString=a  RConnTagsString=__new0  NominalVoltage=Vstation  NominalFrequency=frequence  ActivePower=activeA(28,29)/2  InductivePower=reactiveA(28,29)/2  CapacitivePower=0  Setx0=off  InitialVoltage=0  SetiL0=off  InitialCurrent=0  Measurements=None  LoadType=constant Z
  charge distributive 846-848 Y-PQ (2)-B : powerlib/Elements/Series RLC Load  LConnTagsString=a  RConnTagsString=__new0  NominalVoltage=Vstation  NominalFrequency=frequence  ActivePower=activeB(28,29)/2  InductivePower=reactiveB(28,29)/2  CapacitivePower=0  Setx0=off  InitialVoltage=0  SetiL0=off  InitialCurrent=0  Measurements=None  LoadType=constant Z
  charge distributive 846-848 Y-PQ (2)-C : powerlib/Elements/Series RLC Load  LConnTagsString=a  RConnTagsString=__new0  NominalVoltage=Vstation  NominalFrequency=frequence  ActivePower=activeC(28,29)/2  InductivePower=reactiveC(28,29)/2  CapacitivePower=0  Setx0=off  InitialVoltage=0  SetiL0=off  InitialCurrent=0  Measurements=None  LoadType=constant Z
  charge distributive 854-856 Y-PQ (1) : powerlib/Elements/Series RLC Load  LConnTagsString=a  RConnTagsString=__new0  NominalVoltage=Vstation  NominalFrequency=frequence  ActivePower=activeB(17, 18)./2  InductivePower=reactiveB(17, 18)./2  CapacitivePower=0  Setx0=off  InitialVoltage=0  SetiL0=off  InitialCurrent=0  Measurements=None  LoadType=constant PQ
  charge distributive 854-856 Y-PQ (2) : powerlib/Elements/Series RLC Load  LConnTagsString=a  RConnTagsString=__new0  NominalVoltage=Vstation  NominalFrequency=frequence  ActivePower=activeB(17, 18)./2  InductivePower=reactiveB(17, 18)./2  CapacitivePower=0  Setx0=off  InitialVoltage=0  SetiL0=off  InitialCurrent=0  Measurements=None  LoadType=constant PQ
  charge distributive 858-834 D-PQ (1)-A : powerlib/Elements/Series RLC Load  LConnTagsString=a  RConnTagsString=__new0  NominalVoltage=Ustation  NominalFrequency=frequence  ActivePower=activeA(23,25)/2  InductivePower=reactiveA(23,25)/2  CapacitivePower=0  Setx0=off  InitialVoltage=0  SetiL0=off  InitialCurrent=0  Measurements=None  LoadType=constant Z
  charge distributive 858-834 D-PQ (1)-B : powerlib/Elements/Series RLC Load  LConnTagsString=a  RConnTagsString=__new0  NominalVoltage=Ustation  NominalFrequency=frequence  ActivePower=activeB(23,25)/2  InductivePower=reactiveB(23,25)/2  CapacitivePower=0  Setx0=off  InitialVoltage=0  SetiL0=off  InitialCurrent=0  Measurements=None  LoadType=constant Z
  charge distributive 858-834 D-PQ (1)-C : powerlib/Elements/Series RLC Load  LConnTagsString=a  RConnTagsString=__new0  NominalVoltage=Ustation  NominalFrequency=frequence  ActivePower=activeC(23,25)/2  InductivePower=reactiveC(23,25)/2  CapacitivePower=0  Setx0=off  InitialVoltage=0  SetiL0=off  InitialCurrent=0  Measurements=None  LoadType=constant Z
  charge distributive 858-834 D-PQ (2)-A : powerlib/Elements/Series RLC Load  LConnTagsString=a  RConnTagsString=__new0  NominalVoltage=Ustation  NominalFrequency=frequence  ActivePower=activeA(23,25)/2  InductivePower=reactiveA(23,25)/2  CapacitivePower=0  Setx0=off  InitialVoltage=0  SetiL0=off  InitialCurrent=0  Measurements=None  LoadType=constant Z
  charge distributive 858-834 D-PQ (2)-B : powerlib/Elements/Series RLC Load  LConnTagsString=a  RConnTagsString=__new0  NominalVoltage=Ustation  NominalFrequency=frequence  ActivePower=activeB(23,25)/2  InductivePower=reactiveB(23,25)/2  CapacitivePower=0  Setx0=off  InitialVoltage=0  SetiL0=off  InitialCurrent=0  Measurements=None  LoadType=constant Z
  charge distributive 858-834 D-PQ (2)-C : powerlib/Elements/Series RLC Load  LConnTagsString=a  RConnTagsString=__new0  NominalVoltage=Ustation  NominalFrequency=frequence  ActivePower=activeC(23,25)/2  InductivePower=reactiveC(23,25)/2  CapacitivePower=0  Setx0=off  InitialVoltage=0  SetiL0=off  InitialCurrent=0  Measurements=None  LoadType=constant Z
  charge distributive 858-864 Y-PQ (1) : powerlib/Elements/Series RLC Load  LConnTagsString=a  RConnTagsString=__new0  NominalVoltage=Vstation  NominalFrequency=frequence  ActivePower=activeA(23, 24)./2  InductivePower=reactiveA(23, 24)./2  CapacitivePower=0  Setx0=off  InitialVoltage=0  SetiL0=off  InitialCurrent=0  Measurements=None  LoadType=constant PQ
  charge distributive 858-864 Y-PQ (2) : powerlib/Elements/Series RLC Load  LConnTagsString=a  RConnTagsString=__new0  NominalVoltage=Vstation  NominalFrequency=frequence  ActivePower=activeA(23, 24)./2  InductivePower=reactiveA(23, 24)./2  CapacitivePower=0  Setx0=off  InitialVoltage=0  SetiL0=off  InitialCurrent=0  Measurements=None  LoadType=constant PQ
  charge distributive 860-836 D-PQ (1)-A : powerlib/Elements/Series RLC Load  LConnTagsString=a  RConnTagsString=__new0  NominalVoltage=Ustation  NominalFrequency=frequence  ActivePower=activeA(30,31)/2  InductivePower=reactiveA(30,31)/2  CapacitivePower=0  Setx0=off  InitialVoltage=0  SetiL0=off  InitialCurrent=0  Measurements=None  LoadType=constant Z
  charge distributive 860-836 D-PQ (1)-B : powerlib/Elements/Series RLC Load  LConnTagsString=a  RConnTagsString=__new0  NominalVoltage=Ustation  NominalFrequency=frequence  ActivePower=activeB(30,31)/2  InductivePower=reactiveB(30,31)/2  CapacitivePower=0  Setx0=off  InitialVoltage=0  SetiL0=off  InitialCurrent=0  Measurements=None  LoadType=constant Z
  charge distributive 860-836 D-PQ (1)-C : powerlib/Elements/Series RLC Load  LConnTagsString=a  RConnTagsString=__new0  NominalVoltage=Ustation  NominalFrequency=frequence  ActivePower=activeC(30,31)/2  InductivePower=reactiveC(30,31)/2  CapacitivePower=0  Setx0=off  InitialVoltage=0  SetiL0=off  InitialCurrent=0  Measurements=None  LoadType=constant Z
  charge distributive 860-836 D-PQ (2)-A : powerlib/Elements/Series RLC Load  LConnTagsString=a  RConnTagsString=__new0  NominalVoltage=Ustation  NominalFrequency=frequence  ActivePower=activeA(30,31)/2  InductivePower=reactiveA(30,31)/2  CapacitivePower=0  Setx0=off  InitialVoltage=0  SetiL0=off  InitialCurrent=0  Measurements=None  LoadType=constant Z
  charge distributive 860-836 D-PQ (2)-B : powerlib/Elements/Series RLC Load  LConnTagsString=a  RConnTagsString=__new0  NominalVoltage=Ustation  NominalFrequency=frequence  ActivePower=activeB(30,31)/2  InductivePower=reactiveB(30,31)/2  CapacitivePower=0  Setx0=off  InitialVoltage=0  SetiL0=off  InitialCurrent=0  Measurements=None  LoadType=constant Z
  charge distributive 860-836 D-PQ (2)-C : powerlib/Elements/Series RLC Load  LConnTagsString=a  RConnTagsString=__new0  NominalVoltage=Ustation  NominalFrequency=frequence  ActivePower=activeC(30,31)/2  InductivePower=reactiveC(30,31)/2  CapacitivePower=0  Setx0=off  InitialVoltage=0  SetiL0=off  InitialCurrent=0  Measurements=None  LoadType=constant Z
  charge distributive 862-838 Y-PQ (1) : powerlib/Elements/Series RLC Load  LConnTagsString=a  RConnTagsString=__new0  NominalVoltage=Vstation  NominalFrequency=frequence  ActivePower=activeB(32, 33)./2  InductivePower=reactiveB(32, 33)./2  CapacitivePower=0  Setx0=off  InitialVoltage=0  SetiL0=off  InitialCurrent=0  Measurements=None  LoadType=constant PQ
  charge distributive 862-838 Y-PQ (2) : powerlib/Elements/Series RLC Load  LConnTagsString=a  RConnTagsString=__new0  NominalVoltage=Vstation  NominalFrequency=frequence  ActivePower=activeB(32, 33)./2  InductivePower=reactiveB(32, 33)./2  CapacitivePower=0  Setx0=off  InitialVoltage=0  SetiL0=off  InitialCurrent=0  Measurements=None  LoadType=constant PQ
  charge ponctuelle 830 DZ-A : powerlib/Elements/Series RLC Load  LConnTagsString=a  RConnTagsString=__new0  NominalVoltage=Ustation  NominalFrequency=frequence  ActivePower=activeA(16,16)  InductivePower=reactiveA(16,16)  CapacitivePower=0  Setx0=off  InitialVoltage=0  SetiL0=off  InitialCurrent=0  Measurements=None  LoadType=constant Z
  charge ponctuelle 830 DZ-B : powerlib/Elements/Series RLC Load  LConnTagsString=a  RConnTagsString=__new0  NominalVoltage=Ustation  NominalFrequency=frequence  ActivePower=activeB(16,16)  InductivePower=reactiveB(16,16)  CapacitivePower=0  Setx0=off  InitialVoltage=0  SetiL0=off  InitialCurrent=0  Measurements=None  LoadType=constant Z
  charge ponctuelle 830 DZ-C : powerlib/Elements/Series RLC Load  LConnTagsString=a  RConnTagsString=__new0  NominalVoltage=Ustation  NominalFrequency=frequence  ActivePower=activeC(16,16)  InductivePower=reactiveC(16,16)  CapacitivePower=0  Setx0=off  InitialVoltage=0  SetiL0=off  InitialCurrent=0  Measurements=None  LoadType=constant Z
  charge ponctuelle 840 YI-A : powerlib/Elements/Series RLC Load  LConnTagsString=a  RConnTagsString=__new0  NominalVoltage=Vstation  NominalFrequency=frequence  ActivePower=activeA(34,34)  InductivePower=reactiveA(34,34)  CapacitivePower=0  Setx0=off  InitialVoltage=0  SetiL0=off  InitialCurrent=0  Measurements=None  LoadType=constant Z
  charge ponctuelle 840 YI-B : powerlib/Elements/Series RLC Load  LConnTagsString=a  RConnTagsString=__new0  NominalVoltage=Vstation  NominalFrequency=frequence  ActivePower=activeB(34,34)  InductivePower=reactiveB(34,34)  CapacitivePower=0  Setx0=off  InitialVoltage=0  SetiL0=off  InitialCurrent=0  Measurements=None  LoadType=constant Z
  charge ponctuelle 840 YI-C : powerlib/Elements/Series RLC Load  LConnTagsString=a  RConnTagsString=__new0  NominalVoltage=Vstation  NominalFrequency=frequence  ActivePower=activeC(34,34)  InductivePower=reactiveC(34,34)  CapacitivePower=0  Setx0=off  InitialVoltage=0  SetiL0=off  InitialCurrent=0  Measurements=None  LoadType=constant Z
  charge ponctuelle 844 Y-Z-A : powerlib/Elements/Series RLC Load  LConnTagsString=a  RConnTagsString=__new0  NominalVoltage=Vstation  NominalFrequency=frequence  ActivePower=activeA(27,27)  InductivePower=reactiveA(27,27)  CapacitivePower=0  Setx0=off  InitialVoltage=0  SetiL0=off  InitialCurrent=0  Measurements=None  LoadType=constant Z
  charge ponctuelle 844 Y-Z-B : powerlib/Elements/Series RLC Load  LConnTagsString=a  RConnTagsString=__new0  NominalVoltage=Vstation  NominalFrequency=frequence  ActivePower=activeB(27,27)  InductivePower=reactiveB(27,27)  CapacitivePower=0  Setx0=off  InitialVoltage=0  SetiL0=off  InitialCurrent=0  Measurements=None  LoadType=constant Z
  charge ponctuelle 844 Y-Z-C : powerlib/Elements/Series RLC Load  LConnTagsString=a  RConnTagsString=__new0  NominalVoltage=Vstation  NominalFrequency=frequence  ActivePower=activeC(27,27)  InductivePower=reactiveC(27,27)  CapacitivePower=0  Setx0=off  InitialVoltage=0  SetiL0=off  InitialCurrent=0  Measurements=None  LoadType=constant Z
  charge ponctuelle 848 D-PQ-A : powerlib/Elements/Series RLC Load  LConnTagsString=a  RConnTagsString=__new0  NominalVoltage=Ustation  NominalFrequency=frequence  ActivePower=activeA(29,29)  InductivePower=reactiveA(29,29)  CapacitivePower=0  Setx0=off  InitialVoltage=0  SetiL0=off  InitialCurrent=0  Measurements=None  LoadType=constant Z
  charge ponctuelle 848 D-PQ-B : powerlib/Elements/Series RLC Load  LConnTagsString=a  RConnTagsString=__new0  NominalVoltage=Ustation  NominalFrequency=frequence  ActivePower=activeB(29,29)  InductivePower=reactiveB(29,29)  CapacitivePower=0  Setx0=off  InitialVoltage=0  SetiL0=off  InitialCurrent=0  Measurements=None  LoadType=constant Z
  charge ponctuelle 848 D-PQ-C : powerlib/Elements/Series RLC Load  LConnTagsString=a  RConnTagsString=__new0  NominalVoltage=Ustation  NominalFrequency=frequence  ActivePower=activeC(29,29)  InductivePower=reactiveC(29,29)/2  CapacitivePower=0  Setx0=off  InitialVoltage=0  SetiL0=off  InitialCurrent=0  Measurements=None  LoadType=constant Z
  charge ponctuelle 860 Y-PQ-A : powerlib/Elements/Series RLC Load  LConnTagsString=a  RConnTagsString=__new0  NominalVoltage=Vstation  NominalFrequency=frequence  ActivePower=activeA(30,30)  InductivePower=reactiveA(30,30)  CapacitivePower=0  Setx0=off  InitialVoltage=0  SetiL0=off  InitialCurrent=0  Measurements=None  LoadType=constant Z
  charge ponctuelle 860 Y-PQ-B : powerlib/Elements/Series RLC Load  LConnTagsString=a  RConnTagsString=__new0  NominalVoltage=Vstation  NominalFrequency=frequence  ActivePower=activeB(30,30)  InductivePower=reactiveB(30,30)  CapacitivePower=0  Setx0=off  InitialVoltage=0  SetiL0=off  InitialCurrent=0  Measurements=None  LoadType=constant Z
  charge ponctuelle 860 Y-PQ-C : powerlib/Elements/Series RLC Load  LConnTagsString=a  RConnTagsString=__new0  NominalVoltage=Vstation  NominalFrequency=frequence  ActivePower=activeC(30,30)  InductivePower=reactiveC(30,30)  CapacitivePower=0  Setx0=off  InitialVoltage=0  SetiL0=off  InitialCurrent=0  Measurements=None  LoadType=constant Z
  charge ponctuelle 890 DI-A : powerlib/Elements/Series RLC Load  LConnTagsString=a  RConnTagsString=__new0  NominalVoltage=Ustation*0.167068273092370  NominalFrequency=frequence  ActivePower=activeA(22,22)  InductivePower=reactiveA(22,22)  CapacitivePower=0  Setx0=off  InitialVoltage=0  SetiL0=off  InitialCurrent=0  Measurements=None  LoadType=constant Z
  charge ponctuelle 890 DI-B : powerlib/Elements/Series RLC Load  LConnTagsString=a  RConnTagsString=__new0  NominalVoltage=Ustation*0.167068273092370  NominalFrequency=frequence  ActivePower=activeB(22,22)  InductivePower=reactiveB(22,22)  CapacitivePower=0  Setx0=off  InitialVoltage=0  SetiL0=off  InitialCurrent=0  Measurements=None  LoadType=constant Z
  charge ponctuelle 890 DI-C : powerlib/Elements/Series RLC Load  LConnTagsString=a  RConnTagsString=__new0  NominalVoltage=Ustation*0.167068273092370  NominalFrequency=frequence  ActivePower=activeC(22,22)  InductivePower=reactiveC(22,22)  CapacitivePower=0  Setx0=off  InitialVoltage=0  SetiL0=off  InitialCurrent=0  Measurements=None  LoadType=constant Z
  charge ponctuelle capacitive 844 Y-Z-A : powerlib/Elements/Series RLC Load  LConnTagsString=a  RConnTagsString=__new0  NominalVoltage=Vstation  NominalFrequency=frequence  ActivePower=0  InductivePower=0  CapacitivePower=Qc844(1, 1)  Setx0=off  InitialVoltage=0  SetiL0=off  InitialCurrent=0  Measurements=None  LoadType=constant Z
  charge ponctuelle capacitive 844 Y-Z-B : powerlib/Elements/Series RLC Load  LConnTagsString=a  RConnTagsString=__new0  NominalVoltage=Vstation  NominalFrequency=frequence  ActivePower=0  InductivePower=0  CapacitivePower=Qc844(1, 2)  Setx0=off  InitialVoltage=0  SetiL0=off  InitialCurrent=0  Measurements=None  LoadType=constant Z
  charge ponctuelle capacitive 844 Y-Z-C : powerlib/Elements/Series RLC Load  LConnTagsString=a  RConnTagsString=__new0  NominalVoltage=Vstation  NominalFrequency=frequence  ActivePower=0  InductivePower=0  CapacitivePower=Qc844(1, 3)  Setx0=off  InitialVoltage=0  SetiL0=off  InitialCurrent=0  Measurements=None  LoadType=constant Z
  charge ponctuelle capacitive 848 Y-Z-A : powerlib/Elements/Series RLC Load  LConnTagsString=a  RConnTagsString=__new0  NominalVoltage=Vstation  NominalFrequency=frequence  ActivePower=0  InductivePower=0  CapacitivePower=Qc848(1, 1)  Setx0=off  InitialVoltage=0  SetiL0=off  InitialCurrent=0  Measurements=None  LoadType=constant Z
  charge ponctuelle capacitive 848 Y-Z-B : powerlib/Elements/Series RLC Load  LConnTagsString=a  RConnTagsString=__new0  NominalVoltage=Vstation  NominalFrequency=frequence  ActivePower=0  InductivePower=0  CapacitivePower=Qc848(1, 2)  Setx0=off  InitialVoltage=0  SetiL0=off  InitialCurrent=0  Measurements=None  LoadType=constant Z
  charge ponctuelle capacitive 848 Y-Z-C : powerlib/Elements/Series RLC Load  LConnTagsString=a  RConnTagsString=__new0  NominalVoltage=Vstation  NominalFrequency=frequence  ActivePower=0  InductivePower=0  CapacitivePower=Qc848(1, 3)  Setx0=off  InitialVoltage=0  SetiL0=off  InitialCurrent=0  Measurements=None  LoadType=constant Z
  ligne 800-802 : powerlib/Elements/Distributed Parameters Line  Phases=3  Frequency=frequence  Resistance=R_300  Inductance=L_300  Capacitance=C_300  Length=Ltot_800_802  x1=[841.740640202652 17597.8209179522 17515.3839283628;376.991118430775 376.991118430775 376.991118430775;1.94160573810257 0.298080075052811 1.87234868535801]  x2=[850.183665430956 17571.8848498328 17489.0043571788;376.991118430775 376.991118430775 376.991118430775;1.95149970714428 0.297360219216009 1.87152220315872]  x3=[9.8690741193051 11.3104925296039 7.70039823989951;376.991118430775 376.991118430775 376.991118430775;1.8087693660521 0.876021611970401 -2.98867694065345]  x4=[7.84662556244415 95.9536172602425 86.3406203210247;376.991118430775 376.991118430775 376.991118430775;-1.36849343678115 0.232633773061638 1.78305984931854]  x5=3.46223763231864e-06  V1=ones(3,3)  V2=ones(3,3)  I1=ones(3,3)  I2=ones(3,3)  nHarmo=1  Measurements=None
  ligne 802-806 : powerlib/Elements/Distributed Parameters Line  Phases=3  Frequency=frequence  Resistance=R_300  Inductance=L_300  Capacitance=C_300  Length=Ltot_802_806  x1=[850.183665430956 17571.8848498328 17489.0043571788;376.991118430775 376.991118430775 376.991118430775;1.9519297257147 0.297726719842833 1.87188156756628]  x2=[855.754123927847 17554.7072923756 17471.9050286117;376.991118430775 376.991118430775 376.991118430775;1.95909007056772 0.297253200646118 1.87132414390253]  x3=[10.213742673881 11.8016325712392 7.04309462614517;376.991118430775 376.991118430775 376.991118430775;1.8628011373405 0.85425864515553 -3.12837599729856]  x4=[8.16062680457256 95.3229415670104 85.3303985035144;376.991118430775 376.991118430775 376.991118430775;-1.30210214170497 0.231605767939526 1.79199650192909]  x5=2.32157794725242e-06  V1=ones(3,3)  V2=ones(3,3)  I1=ones(3,3)  I2=ones(3,3)  nHarmo=1  Measurements=None
  ligne 806-808(1) : powerlib/Elements/Distributed Parameters Line  Phases=3  Frequency=frequence  Resistance=R_300  Inductance=L_300  Capacitance=C_300  Length=disdef  x1=[855.754123927847 17554.7072923756 17471.9050286117;376.991118430775 376.991118430775 376.991118430775;1.94365999245258 0.284102295801276 1.8584293033961]  x2=[965.237623788486 17237.7181129311 17163.7114806022;376.991118430775 376.991118430775 376.991118430775;2.07208837299579 0.275438288751485 1.84791959437163]  x3=[10.5179067457503 11.9740432316221 6.42689812109088;376.991118430775 376.991118430775 376.991118430775;1.89698984573436 0.830164467971759 2.9984020745509]  x4=[8.35333728143084 92.6909711360465 82.8173114927329;376.991118430775 376.991118430775 376.991118430775;-1.27236854802587 0.204444118636162 1.77542231697895]  x5=4.32511313525697e-05  V1=ones(3,3)  V2=ones(3,3)  I1=ones(3,3)  I2=ones(3,3)  nHarmo=1  Measurements=None
  ligne 806-808(2) : powerlib/Elements/Distributed Parameters Line  Phases=3  Frequency=frequence  Resistance=R_300  Inductance=L_300  Capacitance=C_300  Length=Ltot_806_808-disdef  x1=[855.754123927847 17554.7072923756 17471.9050286117;376.991118430775 376.991118430775 376.991118430775;1.94365999245258 0.284102295801276 1.8584293033961]  x2=[965.237623788486 17237.7181129311 17163.7114806022;376.991118430775 376.991118430775 376.991118430775;2.07208837299579 0.275438288751485 1.84791959437163]  x3=[10.5179067457503 11.9740432316221 6.42689812109088;376.991118430775 376.991118430775 376.991118430775;1.89698984573436 0.830164467971759 2.9984020745509]  x4=[8.35333728143084 92.6909711360465 82.8173114927329;376.991118430775 376.991118430775 376.991118430775;-1.27236854802587 0.204444118636162 1.77542231697895]  x5=4.32511313525697e-05  V1=ones(3,3)  V2=ones(3,3)  I1=ones(3,3)  I2=ones(3,3)  nHarmo=1  Measurements=None
  ligne 808-810 : powerlib/Elements/Distributed Parameters Line  Phases=1  Frequency=frequence  Resistance=R_303  Inductance=L_303  Capacitance=C_303  Length=Ltot_808_810  x1=[14121.8857902631;376.991118430775;-2.11609281146975]  x2=[14119.8111214169;376.991118430775;-2.11610360523278]  x3=[23.179608705473;376.991118430775;-2.10715523907707]  x4=[24.2670221088205;376.991118430775;-2.12733612307997]  x5=7.30496713110932e-06  V1=ones(3,3)  V2=ones(3,3)  I1=ones(3,3)  I2=ones(3,3)  nHarmo=1  Measurements=None
  ligne 808-812 : powerlib/Elements/Distributed Parameters Line  Phases=3  Frequency=frequence  Resistance=R_300  Inductance=L_300  Capacitance=C_300  Length=Ltot_808_812  x1=[965.237623788486 17237.7181129311 17163.7114806022;376.991118430775 376.991118430775 376.991118430775;2.06942225785918 0.273165984865179 1.84569153504478]  x2=[1096.77467131991 16870.4492766013 16809.5731029754;376.991118430775 376.991118430775 376.991118430775;2.19282469684806 0.263366146597648 1.83304927474484]  x3=[10.4631107304982 11.9667007839268 5.71326120551019;376.991118430775 376.991118430775 376.991118430775;1.97678152360496 0.876443315554198 3.04904573205666]  x4=[8.03316480097524 90.8648303340973 81.6201097655523;376.991118430775 376.991118430775 376.991118430775;-1.21031638364248 0.183993068309503 1.7657461566632]  x5=5.03232213999802e-05  V1=ones(3,3)  V2=ones(3,3)  I1=ones(3,3)  I2=ones(3,3)  nHarmo=1  Measurements=None
  ligne 812-814 : powerlib/Elements/Distributed Parameters Line  Phases=3  Frequency=frequence  Resistance=R_300  Inductance=L_300  Capacitance=C_300  Length=Ltot_812_814  x1=[1096.77467131991 16870.4492766013 16809.5731029754;376.991118430775 376.991118430775 376.991118430775;2.19675557248592 0.266716393504022 1.83633428821156]  x2=[1210.28752190253 16577.2957340906 16527.7452137713;376.991118430775 376.991118430775 376.991118430775;2.27483330242003 0.258916415553206 1.82615119410095]  x3=[10.6095884600756 11.37483507733 5.62101549988128;376.991118430775 376.991118430775 376.991118430775;1.99940817982855 0.954659662737169 -3.08365634123181]  x4=[7.94062072660981 90.3703015595994 81.1994467259617;376.991118430775 376.991118430775 376.991118430775;-1.22198812266746 0.17540388638646 1.75702830853253]  x5=3.98962499259043e-05  V1=ones(3,3)  V2=ones(3,3)  I1=ones(3,3)  I2=ones(3,3)  nHarmo=1  Measurements=None
  ligne 814-850 : powerlib/Elements/Distributed Parameters Line  Phases=3  Frequency=frequence  Resistance=R_301  Inductance=L_301  Capacitance=C_301  Length=Ltot_814_850  x1=[305.590150304608 16581.0877635211 16545.4852487804;376.991118430775 376.991118430775 376.991118430775;-1.75920576763049 0.270184679049474 1.83571759081233]  x2=[305.580968021365 16580.9443376898 16545.3488009621;376.991118430775 376.991118430775 376.991118430775;-1.75941525800993 0.270182479981793 1.83571455586298]  x3=[9.69772117355039 10.1140491769548 5.71937369479962;376.991118430775 376.991118430775 376.991118430775;2.00598635004601 1.09792782796234 -2.94040624656718]  x4=[10.2468510309043 90.0252015901766 80.1723866220812;376.991118430775 376.991118430775 376.991118430775;-1.1736539004772 0.187353592478204 1.76446008827778]  x5=1.37899021776565e-08  V1=ones(3,3)  V2=ones(3,3)  I1=ones(3,3)  I2=ones(3,3)  nHarmo=1  Measurements=None
  ligne 816-818 : powerlib/Elements/Distributed Parameters Line  Phases=1  Frequency=frequence  Resistance=R_302  Inductance=L_302  Capacitance=C_302  Length=Ltot_816_818  x1=[13178.2972737927;376.991118430775;-0.0225660272285814]  x2=[13164.0317240068;376.991118430775;-0.0222802904737531]  x3=[15.180574421387;376.991118430775;0.673659053489925]  x4=[34.148135176154;376.991118430775;-0.312035325589182]  x5=2.15222153587129e-06  V1=ones(3,3)  V2=ones(3,3)  I1=ones(3,3)  I2=ones(3,3)  nHarmo=1  Measurements=None
  ligne 816-824 : powerlib/Elements/Distributed Parameters Line  Phases=3  Frequency=frequence  Resistance=R_301  Inductance=L_301  Capacitance=C_301  Length=Ltot_816_824  x1=[305.30297121809 16576.4980290699 16541.1188514707;376.991118430775 376.991118430775 376.991118430775;-1.7712182457757 0.265792732287339 1.8313666558972]  x2=[281.937100311529 16462.9288973514 16407.6879740113;376.991118430775 376.991118430775 376.991118430775;-1.80306449120352 0.26218312985224 1.8288610627025]  x3=[3.49548115213852 12.574150782433 7.84453783248638;376.991118430775 376.991118430775 376.991118430775;0.869047112979662 0.101627079527652 3.01525828728126]  x4=[4.07193268701252 83.1302687022051 76.9268082299161;376.991118430775 376.991118430775 376.991118430775;-2.1995672465348 0.285956357736995 1.73327841289057]  x5=1.40794901233873e-05  V1=ones(3,3)  V2=ones(3,3)  I1=ones(3,3)  I2=ones(3,3)  nHarmo=1  Measurements=None
  ligne 818-820 : powerlib/Elements/Distributed Parameters Line  Phases=1  Frequency=frequence  Resistance=R_302  Inductance=L_302  Capacitance=C_302  Length=Ltot_818_820  x1=[13164.0317240068;376.991118430775;-0.0443153481801826]  x2=[12801.5190786927;376.991118430775;-0.0365286168237435]  x3=[14.8868480949058;376.991118430775;0.563085915248821]  x4=[31.441882262828;376.991118430775;-0.328756734915763]  x5=6.06020274574283e-05  V1=ones(3,3)  V2=ones(3,3)  I1=ones(3,3)  I2=ones(3,3)  nHarmo=1  Measurements=None
  ligne 820-822 : powerlib/Elements/Distributed Parameters Line  Phases=1  Frequency=frequence  Resistance=R_302  Inductance=L_302  Capacitance=C_302  Length=Ltot_820_822  x1=[12801.5190786927;376.991118430775;-0.0202016070115506]  x2=[12755.3289672225;376.991118430775;-0.0191288049683156]  x3=[17.7037526767385;376.991118430775;0.207497918998471]  x4=[25.7894625819058;376.991118430775;-0.180375716934438]  x5=1.72932888320886e-05  V1=ones(3,3)  V2=ones(3,3)  I1=ones(3,3)  I2=ones(3,3)  nHarmo=1  Measurements=None
  ligne 824-826 : powerlib/Elements/Distributed Parameters Line  Phases=1  Frequency=frequence  Resistance=R_303  Inductance=L_303  Capacitance=C_303  Length=Ltot_824_826  x1=[13571.2556256492;376.991118430775;-2.15417134432333]  x2=[13568.6004769129;376.991118430775;-2.15417805286552]  x3=[21.5389646596412;376.991118430775;-2.12525241541556]  x4=[24.1569679382857;376.991118430775;-2.18132244926038]  x5=3.81358552847368e-06  V1=ones(3,3)  V2=ones(3,3)  I1=ones(3,3)  I2=ones(3,3)  nHarmo=1  Measurements=None
  ligne 824-828 : powerlib/Elements/Distributed Parameters Line  Phases=3  Frequency=frequence  Resistance=R_301  Inductance=L_301  Capacitance=C_301  Length=Ltot_824_828  x1=[281.937100311529 16462.9288973514 16407.6879740113;376.991118430775 376.991118430775 376.991118430775;-1.79819333680915 0.266153049394816 1.83276872720967]  x2=[280.957696543769 16454.0273307887 16397.0720252869;376.991118430775 376.991118430775 376.991118430775;-1.80112278588664 0.265876418614781 1.83254137726111]  x3=[2.04423751623597 14.1802813994662 6.63973419457376;376.991118430775 376.991118430775 376.991118430775;1.19861428109399 0.155925662268872 2.89419846479566]  x4=[2.65387018869564 81.7100253858249 76.5841876334169;376.991118430775 376.991118430775 376.991118430775;-1.90995150185396 0.284873970015042 1.75670276330336]  x5=1.15835178292315e-06  V1=ones(3,3)  V2=ones(3,3)  I1=ones(3,3)  I2=ones(3,3)  nHarmo=1  Measurements=None
  ligne 828-830 : powerlib/Elements/Distributed Parameters Line  Phases=3  Frequency=frequence  Resistance=R_301  Inductance=L_301  Capacitance=C_301  Length=Ltot_828_830  x1=[280.957696543769 16454.0273307887 16397.0720252869;376.991118430775 376.991118430775 376.991118430775;-1.81131218035085 0.257572211247173 1.82436739387365]  x2=[256.243398220781 16238.4965735678 16139.329330929;376.991118430775 376.991118430775 376.991118430775;-1.88724946749785 0.25080033161402 1.81885263799788]  x3=[2.10415542579107 13.9614494686595 6.59434458760507;376.991118430775 376.991118430775 376.991118430775;1.13432675855298 0.136727598278497 2.89057713006224]  x4=[2.68060544186237 79.9874612280468 75.1352580391864;376.991118430775 376.991118430775 376.991118430775;-1.97387570953247 0.269563496682462 1.74015210528101]  x5=2.81865600511299e-05  V1=ones(3,3)  V2=ones(3,3)  I1=ones(3,3)  I2=ones(3,3)  nHarmo=1  Measurements=None
  ligne 830-854 : powerlib/Elements/Distributed Parameters Line  Phases=3  Frequency=frequence  Resistance=R_301  Inductance=L_301  Capacitance=C_301  Length=Ltot_830_854  x1=[256.243398220781 16238.4965735678 16139.329330929;376.991118430775 376.991118430775 376.991118430775;-1.87689371557299 0.259240117877425 1.82716007417534]  x2=[255.614783785295 16233.1915950729 16133.0834236299;376.991118430775 376.991118430775 376.991118430775;-1.87878096621225 0.259070851823889 1.82701922774134]  x3=[2.07485448627276 14.7246182272078 6.6423344462303;376.991118430775 376.991118430775 376.991118430775;1.07193884715797 0.145304129376725 2.71264840500453]  x4=[2.62559783287676 79.9033175943928 74.2983699750676;376.991118430775 376.991118430775 376.991118430775;-2.02909534326918 0.279961965414028 1.75769942679107]  x5=7.17074913238139e-07  V1=ones(3,3)  V2=ones(3,3)  I1=ones(3,3)  I2=ones(3,3)  nHarmo=1  Measurements=None
  ligne 832-858 : powerlib/Elements/Distributed Parameters Line  Phases=3  Frequency=frequence  Resistance=R_301  Inductance=L_301  Capacitance=C_301  Length=Ltot_832_858  x1=[215.567225257912 15856.4921314291 15691.5204020499;376.991118430775 376.991118430775 376.991118430775;-2.02467320277663 0.245352514777246 1.81516592623891]  x2=[210.858605824763 15825.7676894922 15652.7701716957;376.991118430775 376.991118430775 376.991118430775;-2.03896628459802 0.243657949276636 1.81378377765116]  x3=[1.53639469553167 24.3421618175207 12.9856570508759;376.991118430775 376.991118430775 376.991118430775;0.821336700645947 -0.0384511651549761 1.7852681515769]  x4=[1.98652278805152 68.8882332136614 62.898560128962;376.991118430775 376.991118430775 376.991118430775;-2.25391976190191 0.341929323227552 1.81927112596478]  x5=6.7570520670517e-06  V1=ones(3,3)  V2=ones(3,3)  I1=ones(3,3)  I2=ones(3,3)  nHarmo=1  Measurements=None
  ligne 834-842 : powerlib/Elements/Distributed Parameters Line  Phases=3  Frequency=frequence  Resistance=R_301  Inductance=L_301  Capacitance=C_301  Length=Ltot_834_842  x1=[205.095656726148 15790.7571953981 15608.0597581365;376.991118430775 376.991118430775 376.991118430775;-2.05296257626516 0.243610474380701 1.81405852304482]  x2=[204.856226645832 15789.9132878075 15607.2428443859;376.991118430775 376.991118430775 376.991118430775;-2.05334324633871 0.243517999924749 1.81396906967107]  x3=[1.19594043304138 33.5364262498273 25.6172864516069;376.991118430775 376.991118430775 376.991118430775;0.487890203340123 -0.057826380254029 1.48403591691253]  x4=[1.58554276919261 60.7330566521454 52.1964994414498;376.991118430775 376.991118430775 376.991118430775;-2.49350732731817 0.408134189903033 1.97363131850155]  x5=3.86117260974383e-07  V1=ones(3,3)  V2=ones(3,3)  I1=ones(3,3)  I2=ones(3,3)  nHarmo=1  Measurements=None
  ligne 834-860 : powerlib/Elements/Distributed Parameters Line  Phases=3  Frequency=frequence  Resistance=R_301  Inductance=L_301  Capacitance=C_301  Length=Ltot_834_860  x1=[205.095656726148 15790.7571953981 15608.0597581365;376.991118430775 376.991118430775 376.991118430775;-2.05386714495739 0.242873264134802 1.8133328734992]  x2=[204.937495263295 15785.8113137041 15601.0520525864;376.991118430775 376.991118430775 376.991118430775;-2.05617185529598 0.242885685099382 1.81336792012554]  x3=[0.198564479379918 39.815179299363 30.2167690308728;376.991118430775 376.991118430775 376.991118430775;1.99115471342757 0.321121063848725 1.98617518255077]  x4=[0.591048460266189 52.2154245150751 46.2069600578928;376.991118430775 376.991118430775 376.991118430775;-1.78814509548912 0.182490245581514 1.69996147371272]  x5=2.78556023988662e-06  V1=ones(3,3)  V2=ones(3,3)  I1=ones(3,3)  I2=ones(3,3)  nHarmo=1  Measurements=None
  ligne 836-840 : powerlib/Elements/Distributed Parameters Line  Phases=3  Frequency=frequence  Resistance=R_301  Inductance=L_301  Capacitance=C_301  Length=Ltot_836_840  x1=[204.955732056564 15782.7567756014 15598.1444295476;376.991118430775 376.991118430775 376.991118430775;-2.05691483737777 0.243407528105881 1.81383835944637]  x2=[204.953500248908 15782.2516529673 15597.7863843977;376.991118430775 376.991118430775 376.991118430775;-2.05701133818111 0.243414036982697 1.81383860151325]  x3=[0.196143315611683 44.5591397591183 36.8453703805947;376.991118430775 376.991118430775 376.991118430775;-2.16514932115345 0.265678164294178 1.82878577377007]  x4=[0.253343653590607 47.3170805248226 38.8585913938885;376.991118430775 376.991118430775 376.991118430775;-1.9736651848807 0.222087666220542 1.79931622362832]  x5=1.18593158727846e-06  V1=ones(3,3)  V2=ones(3,3)  I1=ones(3,3)  I2=ones(3,3)  nHarmo=1  Measurements=None
  ligne 836-862 : powerlib/Elements/Distributed Parameters Line  Phases=3  Frequency=frequence  Resistance=R_301  Inductance=L_301  Capacitance=C_301  Length=Ltot_836_862  x1=[204.955732056564 15782.7567756014 15598.1444295476;376.991118430775 376.991118430775 376.991118430775;-2.05661331448036 0.243653264854514 1.81408024262825]  x2=[204.959354459901 15782.7597263106 15598.1435446794;376.991118430775 376.991118430775 376.991118430775;-2.05663431614357 0.243653167446436 1.81408006050231]  x3=[0.222068332995121 45.9673918104494 37.8400156042983;376.991118430775 376.991118430775 376.991118430775;-2.1955316869208 0.243014728308665 1.81347912200261]  x4=[0.229695451765694 45.9257528299509 37.8820484884743;376.991118430775 376.991118430775 376.991118430775;-1.92249994337936 0.244173589829072 1.81456380152294]  x5=3.86117260974383e-07  V1=ones(3,3)  V2=ones(3,3)  I1=ones(3,3)  I2=ones(3,3)  nHarmo=1  Measurements=None
  ligne 842-844 : powerlib/Elements/Distributed Parameters Line  Phases=3  Frequency=frequence  Resistance=R_301  Inductance=L_301  Capacitance=C_301  Length=Ltot_842_844  x1=[204.856226645832 15789.9132878075 15607.2428443859;376.991118430775 376.991118430775 376.991118430775;-2.05389950409773 0.243064657991926 1.81352283690451]  x2=[203.586721108746 15785.9495291797 15603.3126424234;376.991118430775 376.991118430775 376.991118430775;-2.0551512862104 0.242616529565345 1.81309381533303]  x3=[1.30376618935831 33.7176837011685 25.6275830538985;376.991118430775 376.991118430775 376.991118430775;0.360994887752863 -0.0617109471616124 1.48589463431319]  x4=[1.66373676529765 60.5344042519253 52.0962104835611;376.991118430775 376.991118430775 376.991118430775;-2.60182115356231 0.410212006585982 1.97176307596713]  x5=1.86163679398363e-06  V1=ones(3,3)  V2=ones(3,3)  I1=ones(3,3)  I2=ones(3,3)  nHarmo=1  Measurements=None
  ligne 844-846 : powerlib/Elements/Distributed Parameters Line  Phases=3  Frequency=frequence  Resistance=R_301  Inductance=L_301  Capacitance=C_301  Length=Ltot_844_846  x1=[203.586721108746 15785.9495291797 15603.3126424234;376.991118430775 376.991118430775 376.991118430775;-2.0563417817881 0.241646293092293 1.8121387938046]  x2=[201.01880296134 15788.2880685834 15606.0477178865;376.991118430775 376.991118430775 376.991118430775;-2.05859173479833 0.240770566336439 1.81135477001535]  x3=[0.936386574203807 44.3272567633346 36.3897248947827;376.991118430775 376.991118430775 376.991118430775;0.291602474474289 -3.10791057745692e-05 1.55707340160433]  x4=[1.28537000181728 49.7833902791171 41.4051600298337;376.991118430775 376.991118430775 376.991118430775;-2.60326911988838 0.454114473120399 2.03358786355676]  x5=5.01952439266698e-06  V1=ones(3,3)  V2=ones(3,3)  I1=ones(3,3)  I2=ones(3,3)  nHarmo=1  Measurements=None
  ligne 846-848 : powerlib/Elements/Distributed Parameters Line  Phases=3  Frequency=frequence  Resistance=R_301  Inductance=L_301  Capacitance=C_301  Length=Ltot_846_848  x1=[201.01880296134 15788.2880685834 15606.0477178865;376.991118430775 376.991118430775 376.991118430775;-2.05697494822774 0.242088223729972 1.81265176431816]  x2=[200.938281056486 15788.775951876 15606.6725941828;376.991118430775 376.991118430775 376.991118430775;-2.05752784004048 0.241967245868424 1.81253174798618]  x3=[0.183102310393208 45.3085371946117 37.5004540184606;376.991118430775 376.991118430775 376.991118430775;1.34715880459731 0.0100405827156023 1.53853671187034]  x4=[0.617478762276665 48.9352518195569 40.9261972248505;376.991118430775 376.991118430775 376.991118430775;-1.98023338962386 0.456325838961762 2.06297883135111]  x5=7.30864815415796e-07  V1=ones(3,3)  V2=ones(3,3)  I1=ones(3,3)  I2=ones(3,3)  nHarmo=1  Measurements=None
  ligne 850-816 : powerlib/Elements/Distributed Parameters Line  Phases=3  Frequency=frequence  Resistance=R_301  Inductance=L_301  Capacitance=C_301  Length=Ltot_850_816  x1=[305.580968021365 16580.9443376898 16545.3488009621;376.991118430775 376.991118430775 376.991118430775;-1.75957121812928 0.270055374766982 1.83558944387235]  x2=[305.30297121809 16576.4980290699 16541.1188514707;376.991118430775 376.991118430775 376.991118430775;-1.76607156183715 0.26998720437608 1.83549535158781]  x3=[9.69707912998006 10.1101443030904 5.71858794317418;376.991118430775 376.991118430775 376.991118430775;2.00583476855488 1.09808339506385 -2.94006704152684]  x4=[10.2446152206225 89.9971575637186 80.1511751621084;376.991118430775 376.991118430775 376.991118430775;-1.17397305884656 0.187104861122887 1.76421216875058]  x5=4.27486967507352e-07  V1=ones(3,3)  V2=ones(3,3)  I1=ones(3,3)  I2=ones(3,3)  nHarmo=1  Measurements=None
  ligne 852-832 : powerlib/Elements/Distributed Parameters Line  Phases=3  Frequency=frequence  Resistance=R_301  Inductance=L_301  Capacitance=C_301  Length=Ltot_852_832  x1=[215.577393897277 15856.5946083277 15691.6405530236;376.991118430775 376.991118430775 376.991118430775;-2.02208503423361 0.247427553005821 1.81720799004254]  x2=[215.567225257912 15856.4921314291 15691.5204020499;376.991118430775 376.991118430775 376.991118430775;-2.02213105283123 0.247424329778654 1.81720525168609]  x3=[1.95509738568131 13.6626706672608 6.22135757725743;376.991118430775 376.991118430775 376.991118430775;1.06219221112916 0.161879095021265 2.84600903356285]  x4=[2.42526179347021 78.7360971148676 73.172676114069;376.991118430775 376.991118430775 376.991118430775;-2.06828531475356 0.262250405556762 1.74430225917726]  x5=1.37899021776565e-08  V1=ones(3,3)  V2=ones(3,3)  I1=ones(3,3)  I2=ones(3,3)  nHarmo=1  Measurements=None
  ligne 854-852 : powerlib/Elements/Distributed Parameters Line  Phases=3  Frequency=frequence  Resistance=R_301  Inductance=L_301  Capacitance=C_301  Length=Ltot_854_852  x1=[255.614783785295 16233.1915950729 16133.0834236299;376.991118430775 376.991118430775 376.991118430775;-1.89765733932427 0.243686883991347 1.81187650647609]  x2=[215.577393897277 15856.5946083277 15691.6405530236;376.991118430775 376.991118430775 376.991118430775;-2.04122653954852 0.231827506308102 1.80185257839323]  x3=[1.90060120024848 14.126635752912 6.41364835080334;376.991118430775 376.991118430775 376.991118430775;1.02370377381169 0.13840543593108 2.709371602579]  x4=[2.40286159348224 77.0115030050537 71.8753081228787;376.991118430775 376.991118430775 376.991118430775;-2.087441410396 0.246728975363099 1.7286820308077]  x5=5.0788209720309e-05  V1=ones(3,3)  V2=ones(3,3)  I1=ones(3,3)  I2=ones(3,3)  nHarmo=1  Measurements=None
  ligne 854-856 : powerlib/Elements/Distributed Parameters Line  Phases=1  Frequency=frequence  Resistance=R_303  Inductance=L_303  Capacitance=C_303  Length=Ltot_854_856  x1=[13347.905773519;376.991118430775;-2.17296619705026]  x2=[13346.7019196692;376.991118430775;-2.17308532246553]  x3=[22.0347800222733;376.991118430775;-2.18125643914506]  x4=[22.2877684759036;376.991118430775;-2.17595280301919]  x5=2.9363349960162e-05  V1=ones(3,3)  V2=ones(3,3)  I1=ones(3,3)  I2=ones(3,3)  nHarmo=1  Measurements=None
  ligne 858-834 : powerlib/Elements/Distributed Parameters Line  Phases=3  Frequency=frequence  Resistance=R_301  Inductance=L_301  Capacitance=C_301  Length=Ltot_858_834  x1=[210.858605824763 15825.7676894922 15652.7701716957;376.991118430775 376.991118430775 376.991118430775;-2.039449760968 0.243263923110724 1.81339593048023]  x2=[205.095656726148 15790.7571953981 15608.0597581365;376.991118430775 376.991118430775 376.991118430775;-2.05584783847314 0.241259027906711 1.81174395121827]  x3=[1.55001454336174 24.9983993130757 13.4637081598025;376.991118430775 376.991118430775 376.991118430775;0.760812232075544 -0.0414710595847364 1.75943112032084]  x4=[1.98403572614847 68.0357549584316 62.1935785080104;376.991118430775 376.991118430775 376.991118430775;-2.3063138157463 0.343628642111628 1.82258958657583]  x5=8.03951296957375e-06  V1=ones(3,3)  V2=ones(3,3)  I1=ones(3,3)  I2=ones(3,3)  nHarmo=1  Measurements=None
  ligne 858-864 : powerlib/Elements/Distributed Parameters Line  Phases=1  Frequency=frequence  Resistance=R_302  Inductance=L_302  Capacitance=C_302  Length=Ltot_858_864  x1=[12566.4535283135;376.991118430775;-0.0396147110688788]  x2=[12566.3911569914;376.991118430775;-0.0396153951088177]  x3=[21.1093534489329;376.991118430775;-0.038946688311606]  x4=[21.2307856157574;376.991118430775;-0.0410463392045883]  x5=2.03894671819385e-06  V1=ones(3,3)  V2=ones(3,3)  I1=ones(3,3)  I2=ones(3,3)  nHarmo=1  Measurements=None
  ligne 860-836 : powerlib/Elements/Distributed Parameters Line  Phases=3  Frequency=frequence  Resistance=R_301  Inductance=L_301  Capacitance=C_301  Length=Ltot_860_836  x1=[204.937495263295 15785.8113137041 15601.0520525864;376.991118430775 376.991118430775 376.991118430775;-2.05651496755855 0.242606053626799 1.81309267374617]  x2=[204.955732056564 15782.7567756014 15598.1444295476;376.991118430775 376.991118430775 376.991118430775;-2.05786099543516 0.242636423136031 1.81307934670325]  x3=[0.162418557732688 43.1774447535223 35.0971870365322;376.991118430775 376.991118430775 376.991118430775;-2.84749737246039 0.283776252013565 1.84769774594073]  x4=[0.352206206186313 48.6415364943782 40.5672112915057;376.991118430775 376.991118430775 376.991118430775;-1.72428035560214 0.205019237279282 1.7820999962181]  x5=3.69569378361195e-06  V1=ones(3,3)  V2=ones(3,3)  I1=ones(3,3)  I2=ones(3,3)  nHarmo=1  Measurements=None
  ligne 862-838 : powerlib/Elements/Distributed Parameters Line  Phases=1  Frequency=frequence  Resistance=R_304  Inductance=L_304  Capacitance=C_304  Length=Ltot_862_838  x1=[12909.9551295656;376.991118430775;-2.18343918866791]  x2=[12909.989046033;376.991118430775;-2.18344274103598]  x3=[22.5692059979496;376.991118430775;-2.18573319493793]  x4=[22.5692061061137;376.991118430775;-2.18344274241642]  x5=6.08033278760362e-06  V1=ones(3,3)  V2=ones(3,3)  I1=ones(3,3)  I2=ones(3,3)  nHarmo=1  Measurements=None
  ligne 888-890 : powerlib/Elements/Distributed Parameters Line  Phases=3  Frequency=frequence  Resistance=R_300  Inductance=L_300  Capacitance=C_300  Length=Ltot_888_890  x1=[197.513816317699 2480.85861715147 2452.46628722082;376.991118430775 376.991118430775 376.991118430775;2.23072307095141 0.196020291490144 1.76803493528358]  x2=[207.751765028491 2301.33584506266 2266.40814372696;376.991118430775 376.991118430775 376.991118430775;2.26043530303354 0.186054878628668 1.75174275508698]  x3=[2.38196844533367 60.1942992259186 61.0930265996883;376.991118430775 376.991118430775 376.991118430775;1.88080706570588 2.81272047552095 -1.90327370703321]  x4=[1.93245361394254 72.920953562143 71.4937659174087;376.991118430775 376.991118430775 376.991118430775;-1.35065066982004 -0.231971108655233 1.31974190409319]  x5=1.41710191462344e-05  V1=ones(3,3)  V2=ones(3,3)  I1=ones(3,3)  I2=ones(3,3)  nHarmo=1  Measurements=None
  powergui : powerlib/powergui  Priority=1  SimulationMode=Phasor  SolverType=Tustin/Backward Euler (TBE)  SampleTime=50e-6  frequency=frequence  SPID=off  DisableSnubberDevices=off  DisableRonSwitches=off  DisableVfSwitches=off  SwTol=0  DisplayEquations=off  Interpol=off  ExternalGateDelay=off  methode=off  Ts=10  FunctionMessages=off  echomessages=off  HookPort=off  EnableUseOfTLC=off  x0status=blocks  frequencyindice=60  Pbase=100e6  ErrMax=1e-4  Iterations=50  UnitsV=kV  UnitsW=MW  buscounter=0  RestoreLinks=warning  ResistiveCurrentMeasurement=off  Frange=[0:2:500]  Ylog=off  Xlog=on  ShowGrid=off  save=off  variable=ZData  structure=0  ZoomFFT=off  StartTime=0.0  cycles=1  DisplayStyle=1  fundamental=60  FreqAxis=off  MaxFrequency=1000  frequencyindicesteady=1  RmsSteady=1  display=off
  tension du jeu de barre : Subsystem
  wires:
  Ia800_802/1 -> To Workspace/1
  Ib800_802/1 -> To Workspace1/1
  Ic800_802/1 -> To Workspace2/1
  Ia802_806/1 -> To Workspace3/1
  Ib802_806/1 -> To Workspace4/1
  Ic802_806/1 -> To Workspace5/1
  Ia806_808/1 -> To Workspace6/1
  Ib806_808/1 -> To Workspace7/1
  Ic806_808/1 -> To Workspace8/1
  Ia808_812/1 -> To Workspace9/1
  Ib808_812/1 -> To Workspace10/1
  Ic808_812/1 -> To Workspace11/1
  Ib808_810/1 -> To Workspace12/1
  Ia812_814/1 -> To Workspace15/1
  Ib812_814/1 -> To Workspace13/1
  Ic812_814/1 -> To Workspace14/1
  Ia814_850/1 -> To Workspace18/1
  Ib814_850/1 -> To Workspace16/1
  Ic814_850/1 -> To Workspace17/1
  Ia850_816/1 -> To Workspace21/1
  Ib850_816/1 -> To Workspace19/1
  Ic850_816/1 -> To Workspace20/1
  Ia816_824/1 -> To Workspace24/1
  Ib816_824/1 -> To Workspace22/1
  Ic816_824/1 -> To Workspace23/1
  Ia816_818/1 -> To Workspace25/1
  V818/1 -> To Workspace26/1
  Ia818_820/1 -> To Workspace27/1
  V820/1 -> To Workspace28/1
  Ia820_822/1 -> To Workspace29/1
  Ib824_826/1 -> To Workspace30/1
  Ia824_828/1 -> To Workspace31/1
  Ib824_828/1 -> To Workspace32/1
  Ic824_828/1 -> To Workspace33/1
  Ia828_830/1 -> To Workspace36/1
  Ib828_830/1 -> To Workspace34/1
  Ic828_830/1 -> To Workspace35/1
  Ib830_854/1 -> To Workspace37/1
  Ia830_854/1 -> To Workspace39/1
  Ic830_854/1 -> To Workspace38/1
  Ia854_852/1 -> To Workspace42/1
  Ib854_852/1 -> To Workspace40/1
  "Ic854_852 "/1 -> To Workspace41/1
  Ib854_856/1 -> To Workspace43/1
  Ia852_832/1 -> To Workspace46/1
  Ib852_832/1 -> To Workspace44/1
  Ic852_832/1 -> To Workspace45/1
  Ia832_858/1 -> To Workspace49/1
  Ib832_858/1 -> To Workspace47/1
  Ic832_858/1 -> To Workspace48/1
  Ia858_864/1 -> To Workspace50/1
  Ia832_888/1 -> To Workspace53/1
  Ib832_888/1 -> To Workspace51/1
  Ic832_888/1 -> To Workspace52/1
  Ib888_890/1 -> To Workspace54/1
  Ia888_890/1 -> To Workspace56/1
  Ic888_890/1 -> To Workspace55/1
  Ib858_834/1 -> To Workspace57/1
  Ia858_834/1 -> To Workspace59/1
  Ic858_834/1 -> To Workspace58/1
  Ib834_860/1 -> To Workspace60/1
  Ia834_860/1 -> To Workspace62/1
  Ic834_860/1 -> To Workspace61/1
  Ia834_842/1 -> To Workspace65/1
  Ib834_842/1 -> To Workspace63/1
  Ic834_842/1 -> To Workspace64/1
  Ia842_844/1 -> To Workspace68/1
  Ib842_844/1 -> To Workspace66/1
  Ic842_844/1 -> To Workspace67/1
  Ia844_846/1 -> To Workspace71/1
  Ib846_846/1 -> To Workspace69/1
  Ic844_846/1 -> To Workspace70/1
  Ia846_848/1 -> To Workspace74/1
  Ib846_848/1 -> To Workspace72/1
  Ic846_848/1 -> To Workspace73/1
  Ib860_836/1 -> To Workspace75/1
  Ia860_836/1 -> To Workspace77/1
  Ic860_836/1 -> To Workspace76/1
  Ib836_840/1 -> To Workspace78/1
  Ia836_840/1 -> To Workspace80/1
  Ic836_840/1 -> To Workspace79/1
  Ia836_862/1 -> To Workspace83/1
  Ib836_862/1 -> To Workspace81/1
  Ic836_862/1 -> To Workspace82/1
  Ib862_838/1 -> To Workspace84/1
  V810/1 -> To Workspace85/1
  V822/1 -> To Workspace87/1
  V826/1 -> To Workspace89/1
  V856/1 -> To Workspace86/1
  V864/1 -> To Workspace88/1
  V838/1 -> To Workspace90/1
  Ia830_1/1 -> To Workspace91/1
  Ib830_1/1 -> To Workspace92/1
  Ic830_1/1 -> To Workspace93/1
  connections:
  808/RConn2 -- Ib808_810/LConn1 -- Ib808_812/LConn1
  816/RConn1 -- Ia816_818/LConn1 -- Ia816_824/LConn1
  824/RConn2 -- Ib824_826/LConn1 -- Ib824_828/LConn1
  854/RConn2 -- Ib854_856/LConn1 -- Ib854_852/LConn1
  832/RConn1 -- Ia832_888/LConn1 -- Ia832_858/LConn1
  832/RConn2 -- Ib832_888/LConn1 -- Ib832_858/LConn1
  832/RConn3 -- Ic832_888/LConn1 -- Ic832_858/LConn1
  858/RConn1 -- Ia858_864/LConn1 -- Ia858_834/LConn1
  834/RConn1 -- Ia834_860/LConn1 -- Ia834_842/LConn1
  834/RConn2 -- Ib834_860/LConn1 -- Ib834_842/LConn1
  834/RConn3 -- Ic834_860/LConn1 -- Ic834_842/LConn1
  836/RConn1 -- Ia836_840/LConn1 -- Ia836_862/LConn1
  836/RConn2 -- Ib836_840/LConn1 -- Ib836_862/LConn1
  836/RConn3 -- Ic836_840/LConn1 -- Ic836_862/LConn1
  ligne 802-806/RConn1 -- charge distributive 802-806 Y-PQ (2)-A/LConn1 -- 806/LConn1
  ligne 802-806/RConn2 -- charge distributive 802-806 Y-PQ (2)-B/LConn1 -- 806/LConn2
  ligne 802-806/RConn3 -- charge distributive 802-806 Y-PQ (2)-C/LConn1 -- 806/LConn3
  charge distributive 816-824 D-I (2)-C/RConn1 -- 824/LConn2 -- ligne 816-824/RConn2 -- charge distributive 816-824 D-I (2)-B/RConn1
  charge distributive 816-824 D-I (2)-B/LConn1 -- 824/LConn1 -- ligne 816-824/RConn1 -- charge distributive 816-824 D-I (2)-A/LConn1
  charge distributive 816-824 D-I (2)-C/LConn1 -- 824/LConn3 -- ligne 816-824/RConn3 -- charge distributive 816-824 D-I (2)-A/RConn1
  ligne 824-828/RConn1 -- charge distributive 824-828 Y-PQ (2)-A/LConn1 -- 828/LConn1
  ligne 824-828/RConn2 -- charge distributive 824-828 Y-PQ (2)-B/LConn1 -- 828/LConn2
  ligne 824-828/RConn3 -- charge distributive 824-828 Y-PQ (2)-C/LConn1 -- 828/LConn3
  Ib830_1/RConn1 -- charge distributive 828-830 Y-PQ (2)-B/LConn1 -- 830/LConn2
  Ia830_1/RConn1 -- 830/LConn1 -- charge distributive 828-830 Y-PQ (2)-A/LConn1
  Ic830_1/RConn1 -- charge distributive 828-830 Y-PQ (2)-C/LConn1 -- 830/LConn3
  charge distributive 832-858 D-Z (2)-A/LConn1 -- charge distributive 832-858 D-Z (2)-B/LConn1 -- ligne 832-858/RConn1 -- 858/LConn1
  charge distributive 832-858 D-Z (2)-A/RConn1 -- 858/LConn3 -- ligne 832-858/RConn3 -- charge distributive 832-858 D-Z (2)-C/LConn1
  charge distributive 858-834 D-PQ (2)-B/RConn1 -- 834/LConn2 -- ligne 858-834/RConn2 -- charge distributive 858-834 D-PQ (2)-C/RConn1
  charge distributive 858-834 D-PQ (2)-A/LConn1 -- charge distributive 858-834 D-PQ (2)-B/LConn1 -- 834/LConn1 -- ligne 858-834/RConn1
  charge distributive 858-834 D-PQ (2)-A/RConn1 -- 834/LConn3 -- ligne 858-834/RConn3 -- charge distributive 858-834 D-PQ (2)-C/LConn1
  charge distributive 834-860 D-Z (2)-B/RConn1 -- 860/LConn2 -- ligne 834-860/RConn2 -- charge distributive 834-860 D-Z (2)-C/RConn1
  charge distributive 834-860 D-Z (2)-A/LConn1 -- 860/LConn1 -- ligne 834-860/RConn1 -- charge distributive 834-860 D-Z (2)-B/LConn1
  charge distributive 834-860 D-Z (2)-A/RConn1 -- 860/LConn3 -- ligne 834-860/RConn3 -- charge distributive 834-860 D-Z (2)-C/LConn1
  charge distributive 860-836 D-PQ (2)-B/RConn1 -- 836/LConn2 -- ligne 860-836/RConn2 -- charge distributive 860-836 D-PQ (2)-C/RConn1
  charge distributive 860-836 D-PQ (2)-A/RConn1 -- 836/LConn3 -- ligne 860-836/RConn3 -- charge distributive 860-836 D-PQ (2)-C/LConn1
  charge distributive 860-836 D-PQ (2)-A/LConn1 -- 836/LConn1 -- ligne 860-836/RConn1 -- charge distributive 860-836 D-PQ (2)-B/LConn1
  ligne 842-844/RConn2 -- charge distributive 842-844 Y-PQ (2)-B/LConn1 -- 844/LConn2
  ligne 842-844/RConn1 -- charge distributive 842-844 Y-PQ (2)-A/LConn1 -- 844/LConn1
  ligne 842-844/RConn3 -- charge distributive 842-844 Y-PQ (2)-C/LConn1 -- 844/LConn3
  ligne 844-846/RConn2 -- charge distributive 844-846 Y-PQ (2)-B/LConn1 -- 846/LConn2
  ligne 844-846/RConn1 -- charge distributive 844-846 Y-PQ (2)-A/LConn1 -- 846/LConn1
  ligne 844-846/RConn3 -- charge distributive 844-846 Y-PQ (2)-C/LConn1 -- 846/LConn3
  ligne 808-810/LConn1 -- Ib808_810/RConn1 -- charge distributive 808-810 Y-I (1)/LConn1
  Ia816_824/RConn1 -- charge distributive 816-824 D-I (1)-A/LConn1 -- charge distributive 816-824 D-I (1)-B/LConn1 -- ligne 816-824/LConn1
  Ib816_824/RConn1 -- charge distributive 816-824 D-I (1)-B/RConn1 -- charge distributive 816-824 D-I (1)-C/RConn1 -- ligne 816-824/LConn2
  Ic816_824/RConn1 -- ligne 816-824/LConn3 -- charge distributive 816-824 D-I (1)-A/RConn1 -- charge distributive 816-824 D-I (1)-C/LConn1
  ligne 816-818/RConn1 -- Ia818_820/LConn1 -- V818/LConn1
  ligne 818-820/LConn1 -- Ia818_820/RConn1 -- charge distributive 818-820 Y-Z (1)/LConn1
  ligne 820-822/LConn1 -- Ia820_822/RConn1 -- charge distributive 820-822 Y-PQ (1)/LConn1
  ligne 818-820/RConn1 -- charge distributive 818-820 Y-Z (2)/LConn1 -- Ia820_822/LConn1 -- V820/LConn1
  ligne 824-826/LConn1 -- Ib824_826/RConn1 -- charge distributive 824-826 Y-I (1)/LConn1
  Ia824_828/RConn1 -- charge distributive 824-828 Y-PQ (1)-A/LConn1 -- ligne 824-828/LConn1
  Ib824_828/RConn1 -- charge distributive 824-828 Y-PQ (1)-B/LConn1 -- ligne 824-828/LConn2
  Ic824_828/RConn1 -- charge distributive 824-828 Y-PQ (1)-C/LConn1 -- ligne 824-828/LConn3
  ligne 854-856/LConn1 -- Ib854_856/RConn1 -- charge distributive 854-856 Y-PQ (1)/LConn1
  charge distributive 832-858 D-Z (1)-A/LConn1 -- ligne 832-858/LConn1 -- Ia832_858/RConn1 -- charge distributive 832-858 D-Z (1)-B/LConn1
  charge distributive 832-858 D-Z (1)-B/RConn1 -- Ib832_858/RConn1 -- ligne 832-858/LConn2 -- charge distributive 832-858 D-Z (1)-C/RConn1
  charge distributive 832-858 D-Z (1)-A/RConn1 -- ligne 832-858/LConn3 -- Ic832_858/RConn1 -- charge distributive 832-858 D-Z (1)-C/LConn1
  ligne 858-864/LConn1 -- Ia858_864/RConn1 -- charge distributive 858-864 Y-PQ (1)/LConn1
  charge distributive 858-834 D-PQ (1)-A/LConn1 -- charge distributive 858-834 D-PQ (1)-B/LConn1 -- ligne 858-834/LConn1 -- Ia858_834/RConn1
  charge distributive 858-834 D-PQ (1)-B/RConn1 -- Ib858_834/RConn1 -- ligne 858-834/LConn2 -- charge distributive 858-834 D-PQ (1)-C/RConn1
  charge distributive 858-834 D-PQ (1)-A/RConn1 -- Ic858_834/RConn1 -- ligne 858-834/LConn3 -- charge distributive 858-834 D-PQ (1)-C/LConn1
  charge distributive 834-860 D-Z (1)-A/RConn1 -- Ic834_860/RConn1 -- ligne 834-860/LConn3 -- charge distributive 834-860 D-Z (1)-C/LConn1
  charge distributive 834-860 D-Z (1)-B/RConn1 -- ligne 834-860/LConn2 -- Ib834_860/RConn1 -- charge distributive 834-860 D-Z (1)-C/RConn1
  charge distributive 834-860 D-Z (1)-A/LConn1 -- ligne 834-860/LConn1 -- Ia834_860/RConn1 -- charge distributive 834-860 D-Z (1)-B/LConn1
  charge distributive 836-840 D-I (1)-A/LConn1 -- charge distributive 836-840 D-I (1)-B/LConn1 -- ligne 836-840/LConn1 -- Ia836_840/RConn1
  charge distributive 836-840 D-I (1)-B/RConn1 -- ligne 836-840/LConn2 -- Ib836_840/RConn1 -- charge distributive 836-840 D-I (1)-C/RConn1
  charge distributive 836-840 D-I (1)-A/RConn1 -- ligne 836-840/LConn3 -- Ic836_840/RConn1 -- charge distributive 836-840 D-I (1)-C/LConn1
  ligne 862-838/LConn1 -- Ib862_838/RConn1 -- charge distributive 862-838 Y-PQ (1)/LConn1
  Ia802_806/RConn1 -- charge distributive 802-806 Y-PQ (1)-A/LConn1 -- ligne 802-806/LConn1
  Ib802_806/RConn1 -- charge distributive 802-806 Y-PQ (1)-B/LConn1 -- ligne 802-806/LConn2
  Ic802_806/RConn1 -- charge distributive 802-806 Y-PQ (1)-C/LConn1 -- ligne 802-806/LConn3
  charge ponctuelle 830 DZ-A/LConn1 -- charge ponctuelle 830 DZ-B/LConn1 -- ligne 830-854/LConn1 -- Ia830_854/RConn1
  charge ponctuelle 830 DZ-B/RConn1 -- ligne 830-854/LConn2 -- Ib830_854/RConn1 -- charge ponctuelle 830 DZ-C/RConn1
  charge ponctuelle 830 DZ-A/RConn1 -- ligne 830-854/LConn3 -- Ic830_854/RConn1 -- charge ponctuelle 830 DZ-C/LConn1
  Ia842_844/RConn1 -- charge distributive 842-844 Y-PQ (1)-A/LConn1 -- ligne 842-844/LConn1
  Ib842_844/RConn1 -- charge distributive 842-844 Y-PQ (1)-B/LConn1 -- ligne 842-844/LConn2
  Ic842_844/RConn1 -- charge distributive 842-844 Y-PQ (1)-C/LConn1 -- ligne 842-844/LConn3
  Ia844_846/RConn1 -- charge ponctuelle capacitive 844 Y-Z-A/LConn1 -- charge ponctuelle 844 Y-Z-A/LConn1 -- charge distributive 844-846 Y-PQ (1)-A/LConn1 -- ligne 844-846/LConn1
  Ib846_846/RConn1 -- charge ponctuelle capacitive 844 Y-Z-B/LConn1 -- charge ponctuelle 844 Y-Z-B/LConn1 -- charge distributive 844-846 Y-PQ (1)-B/LConn1 -- ligne 844-846/LConn2
  Ic844_846/RConn1 -- charge ponctuelle capacitive 844 Y-Z-C/LConn1 -- charge ponctuelle 844 Y-Z-C/LConn1 -- charge distributive 844-846 Y-PQ (1)-C/LConn1 -- ligne 844-846/LConn3
  Ia846_848/RConn1 -- charge distributive 846-848 Y-PQ (1)-A/LConn1 -- ligne 846-848/LConn1
  Ib846_848/RConn1 -- charge distributive 846-848 Y-PQ (1)-B/LConn1 -- ligne 846-848/LConn2
  Ic846_848/RConn1 -- charge distributive 846-848 Y-PQ (1)-C/LConn1 -- ligne 846-848/LConn3
  charge distributive 860-836 D-PQ (1)-A/LConn1 -- charge ponctuelle 860 Y-PQ-A/LConn1 -- Ia860_836/RConn1 -- ligne 860-836/LConn1 -- charge distributive 860-836 D-PQ (1)-B/LConn1
  charge distributive 860-836 D-PQ (1)-B/RConn1 -- charge ponctuelle 860 Y-PQ-B/LConn1 -- Ib860_836/RConn1 -- ligne 860-836/LConn2 -- charge distributive 860-836 D-PQ (1)-C/RConn1
  charge distributive 860-836 D-PQ (1)-A/RConn1 -- charge ponctuelle 860 Y-PQ-C/LConn1 -- Ic860_836/RConn1 -- ligne 860-836/LConn3 -- charge distributive 860-836 D-PQ (1)-C/LConn1
  charge distributive 836-840 D-I (2)-B/RConn1 -- ligne 836-840/RConn2 -- 840/LConn2 -- charge distributive 836-840 D-I (2)-C/RConn1
  charge distributive 836-840 D-I (2)-A/LConn1 -- charge distributive 836-840 D-I (2)-B/LConn1 -- 840/LConn1 -- ligne 836-840/RConn1
  charge distributive 836-840 D-I (2)-A/RConn1 -- 840/LConn3 -- ligne 836-840/RConn3 -- charge distributive 836-840 D-I (2)-C/LConn1
  848/LConn2 -- charge distributive 846-848 Y-PQ (2)-B/LConn1 -- ligne 846-848/RConn2
  848/LConn1 -- charge distributive 846-848 Y-PQ (2)-A/LConn1 -- ligne 846-848/RConn1
  848/LConn3 -- charge distributive 846-848 Y-PQ (2)-C/LConn1 -- ligne 846-848/RConn3
  ligne 808-810/RConn1 -- charge distributive 808-810 Y-I (2)/LConn1 -- V810/LConn1
  ligne 820-822/RConn1 -- charge distributive 820-822 Y-PQ (2)/LConn1 -- V822/LConn1
  ligne 824-826/RConn1 -- charge distributive 824-826 Y-I (2)/LConn1 -- V826/LConn1
  ligne 854-856/RConn1 -- charge distributive 854-856 Y-PQ (2)/LConn1 -- V856/LConn1
  V864/LConn1 -- charge distributive 858-864 Y-PQ (2)/LConn1 -- ligne 858-864/RConn1
  V838/LConn1 -- charge distributive 862-838 Y-PQ (2)/LConn1 -- ligne 862-838/RConn1
  Ia828_830/RConn1 -- ligne 828-830/LConn1 -- charge distributive 828-830 Y-PQ (1)-A/LConn1
  Ib828_830/RConn1 -- charge distributive 828-830 Y-PQ (1)-B/LConn1 -- ligne 828-830/LConn2
  Ic828_830/RConn1 -- ligne 828-830/LConn3 -- charge distributive 828-830 Y-PQ (1)-C/LConn1
  ligne 800-802/RConn3 -- "802 "/LConn3
  "800 "/LConn1 -- Va/RConn1
  ligne 800-802/RConn2 -- "802 "/LConn2
  "800 "/LConn2 -- Vb/RConn1
  ligne 808-812/RConn1 -- 812/LConn1
  "800 "/LConn3 -- Vc/RConn1
  ligne 800-802/RConn1 -- "802 "/LConn1
  ligne 808-812/RConn2 -- 812/LConn2
  ligne 830-854/RConn3 -- 854/LConn3
  Ia808_812/RConn1 -- ligne 808-812/LConn1
  Ic800_802/LConn1 -- "800 "/RConn3
  Ground/LConn1 -- V818/LConn2
  Ia836_862/RConn1 -- ligne 836-862/LConn1
  ligne 830-854/RConn1 -- 854/LConn1
  ligne 854-852/RConn2 -- 852/LConn2
  Ib816_824/LConn1 -- 816/RConn2
  Ic808_812/RConn1 -- ligne 808-812/LConn3
  Ic836_862/RConn1 -- ligne 836-862/LConn3
  Ic824_828/LConn1 -- 824/RConn3
  ligne 852-832/RConn2 -- 832/LConn2
  XFM-1/RConn3 -- 888/LConn3
  ligne 836-862/RConn3 -- 862/LConn3
  Ib862_838/LConn1 -- 862/RConn2
  Ib854_852/RConn1 -- ligne 854-852/LConn2
  Ic808_812/LConn1 -- 808/RConn3
  Ia816_818/RConn1 -- ligne 816-818/LConn1
  ligne 834-842/RConn2 -- 842/LConn2
  Ib800_802/RConn1 -- ligne 800-802/LConn2
  Ia808_812/LConn1 -- 808/RConn1
  ligne 836-862/RConn2 -- 862/LConn2
  Ib858_834/LConn1 -- 858/RConn2
  Ia834_842/RConn1 -- ligne 834-842/LConn1
  Ic800_802/RConn1 -- ligne 800-802/LConn3
  Ib802_806/LConn1 -- "802 "/RConn2
  Ia854_852/RConn1 -- ligne 854-852/LConn1
  "800 "/RConn1 -- Ia800_802/LConn1
  ligne 834-842/RConn3 -- 842/LConn3
  Ic832_888/RConn1 -- XFM-1/LConn3
  Ib832_888/RConn1 -- XFM-1/LConn2
  "Ic854_852 "/RConn1 -- ligne 854-852/LConn3
  Ib806_808/RConn1 -- ligne 806-808(1)/LConn2
  ligne 852-832/RConn3 -- 832/LConn3
  Ib808_812/RConn1 -- ligne 808-812/LConn2
  ligne 814-850/RConn3 -- 850/LConn3
  ligne 836-862/RConn1 -- 862/LConn1
  ligne 812-814/RConn1 -- 814/LConn1
  ligne 854-852/RConn1 -- 852/LConn1
  ligne 852-832/RConn1 -- 832/LConn1
  Ia832_888/RConn1 -- XFM-1/LConn1
  XFM-1/RConn2 -- 888/LConn2
  ligne 814-850/RConn1 -- 850/LConn1
  XFM-1/RConn1 -- 888/LConn1
  Ground1/LConn1 -- V820/LConn2
  Ic816_824/LConn1 -- 816/RConn3
  ligne 834-842/RConn1 -- 842/LConn1
  "Ic854_852 "/LConn1 -- 854/RConn3
  ligne 814-850/RConn2 -- 850/LConn2
  ligne 812-814/RConn3 -- 814/LConn3
  ligne 850-816/RConn2 -- 816/LConn2
  ligne 812-814/RConn2 -- 814/LConn2
  Ia824_828/LConn1 -- 824/RConn1
  ligne 850-816/RConn1 -- 816/LConn1
  Ic858_834/LConn1 -- 858/RConn3
  Ic802_806/LConn1 -- "802 "/RConn3
  Ia854_852/LConn1 -- 854/RConn1
  Ia800_802/RConn1 -- ligne 800-802/LConn1
  "800 "/RConn2 -- Ib800_802/LConn1
  Ib836_862/RConn1 -- ligne 836-862/LConn2
  ligne 830-854/RConn2 -- 854/LConn2
  ligne 808-812/RConn3 -- 812/LConn3
  ligne 850-816/RConn3 -- 816/LConn3
  ligne 854-852/RConn3 -- 852/LConn3
  Ia812_814/RConn1 -- ligne 812-814/LConn1
  Ic844_846/LConn1 -- 844/RConn3
  852/RConn1 -- Ia852_832/LConn1
  850/RConn2 -- Ib850_816/LConn1
  852/RConn2 -- Ib852_832/LConn1
  Ia852_832/RConn1 -- ligne 852-832/LConn1
  Ic888_890/RConn1 -- ligne 888-890/LConn3
  850/RConn1 -- Ia850_816/LConn1
  Ic846_848/LConn1 -- 846/RConn3
  Ic830_854/LConn1 -- 830/RConn3
  Ic814_850/LConn1 -- 814/RConn3
  Ia850_816/RConn1 -- ligne 850-816/LConn1
  Ic888_890/LConn1 -- 888/RConn3
  Ib846_848/LConn1 -- 846/RConn2
  Ic814_850/RConn1 -- ligne 814-850/LConn3
  Ic852_832/RConn1 -- ligne 852-832/LConn3
  Ib850_816/RConn1 -- ligne 850-816/LConn2
  Ia814_850/RConn1 -- ligne 814-850/LConn1
  844/RConn1 -- Ia844_846/LConn1
  Ic860_836/LConn1 -- 860/RConn3
  Ia846_848/LConn1 -- 846/RConn1
  ligne 888-890/RConn1 -- 890/LConn1
  806/RConn2 -- Ib806_808/LConn1
  890/LConn2 -- ligne 888-890/RConn2
  Ib846_846/LConn1 -- 844/RConn2
  Ib888_890/RConn1 -- ligne 888-890/LConn2
  Ib834_842/RConn1 -- ligne 834-842/LConn2
  "802 "/RConn1 -- Ia802_806/LConn1
  830/RConn1 -- Ia830_854/LConn1
  Ic834_842/RConn1 -- ligne 834-842/LConn3
  Ic806_808/LConn1 -- 806/RConn3
  Ia806_808/RConn1 -- ligne 806-808(1)/LConn1
  Ic812_814/LConn1 -- 812/RConn3
  888/RConn2 -- Ib888_890/LConn1
  Ic812_814/RConn1 -- ligne 812-814/LConn3
  806/RConn1 -- Ia806_808/LConn1
  Ic806_808/RConn1 -- ligne 806-808(1)/LConn3
  812/RConn1 -- Ia812_814/LConn1
  Ic828_830/LConn1 -- 828/RConn3
  Ib812_814/RConn1 -- ligne 812-814/LConn2
  814/RConn2 -- Ib814_850/LConn1
  Ib814_850/RConn1 -- ligne 814-850/LConn2
  Ia814_850/LConn1 -- 814/RConn1
  Ic850_816/LConn1 -- 850/RConn3
  Ic850_816/RConn1 -- ligne 850-816/LConn3
  Ic852_832/LConn1 -- 852/RConn3
  828/RConn2 -- Ib828_830/LConn1
  830/RConn2 -- Ib830_854/LConn1
  860/RConn1 -- Ia860_836/LConn1
  Ia888_890/RConn1 -- ligne 888-890/LConn1
  Ib852_832/RConn1 -- ligne 852-832/LConn2
  Ic842_844/LConn1 -- 842/RConn3
  Ib842_844/LConn1 -- 842/RConn2
  888/RConn1 -- Ia888_890/LConn1
  Ia842_844/LConn1 -- 842/RConn1
  828/RConn1 -- Ia828_830/LConn1
  Ib860_836/LConn1 -- 860/RConn2
  812/RConn2 -- Ib812_814/LConn1
  Ground5/LConn1 -- charge distributive 820-822 Y-PQ (2)/RConn1
  Ground17/LConn1 -- V856/LConn2
  Ground16/LConn1 -- V810/LConn2
  Ground21/LConn1 -- V838/LConn2
  Ground19/LConn1 -- V864/LConn2
  Ground18/LConn1 -- V822/LConn2
  Ground20/LConn1 -- V826/LConn2
  Ground7/LConn1 -- charge distributive 854-856 Y-PQ (2)/RConn1
  Ground2/LConn1 -- charge distributive 818-820 Y-Z (2)/RConn1
  Ground11/LConn1 -- charge distributive 862-838 Y-PQ (2)/RConn1
  Ground3/LConn1 -- charge distributive 818-820 Y-Z (1)/RConn1
  ligne 888-890/RConn3 -- 890/LConn3
  Ground10/LConn1 -- charge distributive 862-838 Y-PQ (1)/RConn1
  Ground8/LConn1 -- charge distributive 858-864 Y-PQ (1)/RConn1
  Ground9/LConn1 -- charge distributive 858-864 Y-PQ (2)/RConn1
  Ground6/LConn1 -- charge distributive 854-856 Y-PQ (1)/RConn1
  Ground4/LConn1 -- charge distributive 820-822 Y-PQ (1)/RConn1
  Ic830_1/LConn1 -- ligne 828-830/RConn3
  ligne 828-830/RConn2 -- Ib830_1/LConn1
  ligne 828-830/RConn1 -- Ia830_1/LConn1
  Ground12/LConn1 -- charge distributive 808-810 Y-I (1)/RConn1
  Ground13/LConn1 -- charge distributive 808-810 Y-I (2)/RConn1
  Ground14/LConn1 -- charge distributive 824-826 Y-I (1)/RConn1
  Ground15/LConn1 -- charge distributive 824-826 Y-I (2)/RConn1
  Va/LConn1 -- Ground22/LConn1 -- Vb/LConn1 -- Vc/LConn1
  Ground23/LConn1 -- charge distributive 802-806 Y-PQ (1)-A/RConn1 -- charge distributive 802-806 Y-PQ (1)-C/RConn1 -- charge distributive 802-806 Y-PQ (1)-B/RConn1
  charge distributive 802-806 Y-PQ (2)-B/RConn1 -- charge distributive 802-806 Y-PQ (2)-A/RConn1 -- charge distributive 802-806 Y-PQ (2)-C/RConn1 -- Ground24/LConn1
  charge distributive 824-828 Y-PQ (1)-B/RConn1 -- charge distributive 824-828 Y-PQ (1)-A/RConn1 -- charge distributive 824-828 Y-PQ (1)-C/RConn1 -- Ground25/LConn1
  charge distributive 824-828 Y-PQ (2)-B/RConn1 -- charge distributive 824-828 Y-PQ (2)-A/RConn1 -- charge distributive 824-828 Y-PQ (2)-C/RConn1 -- Ground26/LConn1
  charge distributive 828-830 Y-PQ (1)-B/RConn1 -- charge distributive 828-830 Y-PQ (1)-A/RConn1 -- charge distributive 828-830 Y-PQ (1)-C/RConn1 -- Ground27/LConn1
  charge distributive 828-830 Y-PQ (2)-B/RConn1 -- charge distributive 828-830 Y-PQ (2)-A/RConn1 -- charge distributive 828-830 Y-PQ (2)-C/RConn1 -- Ground28/LConn1
  charge ponctuelle 890 DI-A/LConn1 -- 890/RConn1 -- charge ponctuelle 890 DI-B/LConn1
  charge ponctuelle 890 DI-B/RConn1 -- charge ponctuelle 890 DI-C/RConn1 -- 890/RConn2
  charge ponctuelle 890 DI-A/RConn1 -- 890/RConn3 -- charge ponctuelle 890 DI-C/LConn1
  charge distributive 832-858 D-Z (2)-B/RConn1 -- 858/LConn2 -- ligne 832-858/RConn2 -- charge distributive 832-858 D-Z (2)-C/RConn1
  Ground29/LConn1 -- charge ponctuelle 840 YI-B/RConn1 -- charge ponctuelle 840 YI-A/RConn1 -- charge ponctuelle 840 YI-C/RConn1
  charge ponctuelle 840 YI-A/LConn1 -- 840/RConn1
  charge ponctuelle 840 YI-B/LConn1 -- 840/RConn2
  charge ponctuelle 840 YI-C/LConn1 -- 840/RConn3
  Ground30/LConn1 -- charge ponctuelle 860 Y-PQ-B/RConn1 -- charge ponctuelle 860 Y-PQ-A/RConn1 -- charge ponctuelle 860 Y-PQ-C/RConn1
  Ground31/LConn1 -- charge distributive 842-844 Y-PQ (1)-B/RConn1 -- charge distributive 842-844 Y-PQ (1)-A/RConn1 -- charge distributive 842-844 Y-PQ (1)-C/RConn1
  Ground32/LConn1 -- charge distributive 842-844 Y-PQ (2)-B/RConn1 -- charge distributive 842-844 Y-PQ (2)-A/RConn1 -- charge distributive 842-844 Y-PQ (2)-C/RConn1
  Ground33/LConn1 -- charge ponctuelle 844 Y-Z-B/RConn1 -- charge ponctuelle 844 Y-Z-A/RConn1 -- charge ponctuelle 844 Y-Z-C/RConn1
  Ground34/LConn1 -- charge ponctuelle capacitive 844 Y-Z-B/RConn1 -- charge ponctuelle capacitive 844 Y-Z-A/RConn1 -- charge ponctuelle capacitive 844 Y-Z-C/RConn1
  Ground35/LConn1 -- charge distributive 844-846 Y-PQ (1)-B/RConn1 -- charge distributive 844-846 Y-PQ (1)-A/RConn1 -- charge distributive 844-846 Y-PQ (1)-C/RConn1
  Ground36/LConn1 -- charge distributive 844-846 Y-PQ (2)-B/RConn1 -- charge distributive 844-846 Y-PQ (2)-A/RConn1 -- charge distributive 844-846 Y-PQ (2)-C/RConn1
  Ground37/LConn1 -- charge distributive 846-848 Y-PQ (1)-B/RConn1 -- charge distributive 846-848 Y-PQ (1)-A/RConn1 -- charge distributive 846-848 Y-PQ (1)-C/RConn1
  Ground38/LConn1 -- charge distributive 846-848 Y-PQ (2)-B/RConn1 -- charge distributive 846-848 Y-PQ (2)-A/RConn1 -- charge distributive 846-848 Y-PQ (2)-C/RConn1
  Ground39/LConn1 -- charge ponctuelle capacitive 848 Y-Z-B/RConn1 -- charge ponctuelle capacitive 848 Y-Z-A/RConn1 -- charge ponctuelle capacitive 848 Y-Z-C/RConn1
  charge ponctuelle 848 D-PQ-A/LConn1 -- charge ponctuelle 848 D-PQ-B/LConn1 -- 848/RConn1 -- charge ponctuelle capacitive 848 Y-Z-A/LConn1
  charge ponctuelle 848 D-PQ-B/RConn1 -- 848/RConn2 -- charge ponctuelle capacitive 848 Y-Z-B/LConn1 -- charge ponctuelle 848 D-PQ-C/RConn1
  charge ponctuelle 848 D-PQ-A/RConn1 -- 848/RConn3 -- charge ponctuelle capacitive 848 Y-Z-C/LConn1 -- charge ponctuelle 848 D-PQ-C/LConn1
  ligne 806-808(2)/RConn2 -- 808/LConn2
  ligne 806-808(2)/LConn2 -- ligne 806-808(1)/RConn2
  ligne 806-808(2)/LConn3 -- ligne 806-808(1)/RConn3
  ligne 806-808(2)/LConn1 -- Breaker/LConn1 -- ligne 806-808(1)/RConn1
  ligne 806-808(2)/RConn1 -- 808/LConn1
  ligne 806-808(2)/RConn3 -- 808/LConn3
  RF1/LConn1 -- Breaker/RConn1
  Ground40/LConn1 -- RF1/RConn1
